simulink model "r2_2f_4x_4a_4k_r366"  (R2012b)
(part 3 of 114)

      mask prompts: storage "Storage medium"; dram_dimm "DRAM dimm"; dram_clock "DRAM clock rate"; nsamples "Number of Samples (2^?)"; data_width "Data width"; offset "Start delay support"; circap "Circular capture support"; value "Extra value capture support"; use_dsp48 "Use DSP48s to implement counters"
      mask help:
      | Standard snap block, but with the following optional extras;
      |  1) Optionally delay the fabric trigger by a user-specified number of valids.
      |  2) Capture continuously after a trigger until a stop pulse is received. Data is captured into BRAM continuously, with old data being overwritten until a stop command is received. Then stop capturing when memory is filled. This enables you to get some data before and some data after the stop pulse. Use the 'tr_en_cnt' register to determine where you are in your vector. 'Addr' register's MSb now indicates 'busy capturing'.
      |  3) Optionally capture a value on an input port to a register at the same time as the first data sample.
      |  4) Implement counters using DSP48Es to save resources.
      mask init: same as r2_2f_4x_4a_4k_r366/snap_vacc0
      mask TypeOptions storage: bram | dram
      mask Callback storage: snapshot_callback();
      mask TypeOptions dram_dimm: 1 | 2 | 3 | 4
      mask TypeOptions dram_clock: 200 | 250 | 266 | 300 | 333
      mask TypeOptions data_width: 8 | 16 | 32 | 64 | 128
  snap_xeng2 : Subsystem  Tag=casper:snapshot  AncestorBlock=casper_library_scopes/snapshot  mask(snapshot){storage=bram, dram_dimm=1, dram_clock=200, nsamples=11, data_width=32, offset=on, circap=off, value=off, use_dsp48=on}
      mask prompts: storage "Storage medium"; dram_dimm "DRAM dimm"; dram_clock "DRAM clock rate"; nsamples "Number of Samples (2^?)"; data_width "Data width"; offset "Start delay support"; circap "Circular capture support"; value "Extra value capture support"; use_dsp48 "Use DSP48s to implement counters"
      mask help:
      | Standard snap block, but with the following optional extras;
      |  1) Optionally delay the fabric trigger by a user-specified number of valids.
      |  2) Capture continuously after a trigger until a stop pulse is received. Data is captured into BRAM continuously, with old data being overwritten until a stop command is received. Then stop capturing when memory is filled. This enables you to get some data before and some data after the stop pulse. Use the 'tr_en_cnt' register to determine where you are in your vector. 'Addr' register's MSb now indicates 'busy capturing'.
      |  3) Optionally capture a value on an input port to a register at the same time as the first data sample.
      |  4) Implement counters using DSP48Es to save resources.
      mask init: same as r2_2f_4x_4a_4k_r366/snap_vacc0
      mask TypeOptions storage: bram | dram
      mask Callback storage: snapshot_callback();
      mask TypeOptions dram_dimm: 1 | 2 | 3 | 4
      mask TypeOptions dram_clock: 200 | 250 | 266 | 300 | 333
      mask TypeOptions data_width: 8 | 16 | 32 | 64 | 128
  snap_xeng3 : Subsystem  Tag=casper:snapshot  AncestorBlock=casper_library_scopes/snapshot  mask(snapshot){storage=bram, dram_dimm=1, dram_clock=200, nsamples=11, data_width=32, offset=on, circap=off, value=off, use_dsp48=on}
      mask prompts: storage "Storage medium"; dram_dimm "DRAM dimm"; dram_clock "DRAM clock rate"; nsamples "Number of Samples (2^?)"; data_width "Data width"; offset "Start delay support"; circap "Circular capture support"; value "Extra value capture support"; use_dsp48 "Use DSP48s to implement counters"
      mask help:
      | Standard snap block, but with the following optional extras;
      |  1) Optionally delay the fabric trigger by a user-specified number of valids.
      |  2) Capture continuously after a trigger until a stop pulse is received. Data is captured into BRAM continuously, with old data being overwritten until a stop command is received. Then stop capturing when memory is filled. This enables you to get some data before and some data after the stop pulse. Use the 'tr_en_cnt' register to determine where you are in your vector. 'Addr' register's MSb now indicates 'busy capturing'.
      |  3) Optionally capture a value on an input port to a register at the same time as the first data sample.
      |  4) Implement counters using DSP48Es to save resources.
      mask init: same as r2_2f_4x_4a_4k_r366/snap_vacc0
      mask TypeOptions storage: bram | dram
      mask Callback storage: snapshot_callback();
      mask TypeOptions dram_dimm: 1 | 2 | 3 | 4
      mask TypeOptions dram_clock: 200 | 250 | 266 | 300 | 333
      mask TypeOptions data_width: 8 | 16 | 32 | 64 | 128
  spead_unpack0 : Subsystem  Tag=casper:spead_unpack  AncestorBlock=casper_library_communications/spead_unpack  mask(spead_unpack_mask){payload_length=128, header_ids=[hex2dec('1600'),hex2dec('4101'),hex2dec('4102'), hex2dec('4103')], spead_msw=64, spead_lsw=48, spead_version=4, combine_errors=on}
      mask prompts: payload_length "Payload length in 64-bit words"; header_ids "SPEAD header IDs (decimal)"; spead_msw "SPEAD Flavour (MSw)"; spead_lsw "SPEAD Flavour (LSw)"; spead_version "SPEAD version"; combine_errors "Combine error flags"
      mask help: This block receives a 64-bit-word stream that contains a SPEAD stream. It checks the SPEAD headers are being correctly received. It presents the user with all headers on the first valid cycle of data along with a flag to indicate a header or packet-length error.
      mask init:
      | spead_unpack_init(gcb)
  spead_unpack1 : Subsystem  Tag=casper:spead_unpack  AncestorBlock=casper_library_communications/spead_unpack  mask(spead_unpack_mask){payload_length=128, header_ids=[hex2dec('1600'),hex2dec('4101'),hex2dec('4102'), hex2dec('4103')], spead_msw=64, spead_lsw=48, spead_version=4, combine_errors=on}
      mask prompts: payload_length "Payload length in 64-bit words"; header_ids "SPEAD header IDs (decimal)"; spead_msw "SPEAD Flavour (MSw)"; spead_lsw "SPEAD Flavour (LSw)"; spead_version "SPEAD version"; combine_errors "Combine error flags"
      mask help: This block receives a 64-bit-word stream that contains a SPEAD stream. It checks the SPEAD headers are being correctly received. It presents the user with all headers on the first valid cycle of data along with a flag to indicate a header or packet-length error.
      mask init:
      | spead_unpack_init(gcb)
  status0 : Subsystem  Tag=xps:sw_reg  AncestorBlock=xps_library/software register  mask(swreg){mode=fields of equal size, io_dir=To Processor, io_delay=1, sample_period=1, names=[gbe_down rx_dest_err feng_rx_err fft_err feng_qdr_err feng_chk_err adc_over noise_diode_en vacc_err rx_bad_pkt rx_bad_frame tx_over xeng_bad_dat pack_err rxing_data txing_data], bitwidths=1, arith_types=2, bin_pts=0, sim_port=off, show_format=off}
      mask prompts: io_dir "I/O direction"; io_delay "I/O delay"; sample_period "Sample period"; names "Names [msb ... lsb]:"; bitwidths "Bitwidth:"; arith_types "Type (ufix=0, fix=1, bool=2):"; bin_pts "Binary pt:"; sim_port "Provide sim input/output?"; show_format "Print format string?"
      mask init:
      | swreg_init(gcb)
      settings: AttributesFormatString=16 outputs
      mask TypeOptions mode: one value | fields of equal size | fields of arbitrary size
      mask Callback mode: swreg_cb(gcb);
      mask TypeOptions io_dir: To Processor | From Processor
      mask Callback io_dir:
      | mask_enables = get_param(gcb, 'MaskEnables');
      | mask_names = get_param(gcb, 'MaskNames');
      | if strcmp(get_param(gcb, 'io_dir'), 'To Processor'),
      |     mask_enables{ismember(mask_names, 'sample_period')} = 'off';
      | else
      |     mask_enables{ismember(mask_names, 'sample_period')} = 'on';
      | end
      | set_param(gcb, 'MaskEnables', mask_enables);
      mask Callback bitwidths:
      | blk = gcb;
      | mode = get_param(blk, 'mode');
      | current_widths = eval(get_param(blk, 'bitwidths'));
      | if (strcmp(mode, 'one value') || strcmp(mode, 'fields of equal size')) && (length(current_widths) > 1),
      |     error('Only one width may be specified for this mode.');
      | elseif strcmp(mode, 'fields of arbitrary size')
      |     current_names = textscan(strtrim(strrep(strrep(get_param(blk, 'names'), ']', ''), '[', '')), '%s');
      |     current_names = current_names{1};
      |     numios = length(current_names);
      |     if length(current_widths) ~= numios,
      |         error('%d field names specified, but %d widths?', numios, length(current_widths));
      |     end
      | end
      | total_width = 0;
      | for ctr = 1 : length(current_widths),
      |     total_width = total_width + current_widths(ctr);
      | end
      | if total_width > 32,
      |     error('Total width must be 32 or less, set to %d.', total_width);
      | end
      mask Callback arith_types:
      | blk = gcb;
      | mode = get_param(blk, 'mode');
      | current_types = eval(get_param(blk, 'arith_types'));
      | numios = length(current_types);
      | if (strcmp(mode, 'one value') || strcmp(mode, 'fields of equal size')) && (length(current_types) > 1),
      |     error('Only one type may be specified for this mode.');
      | elseif strcmp(mode, 'fields of arbitrary size')
      |     current_names = textscan(strtrim(strrep(strrep(get_param(blk, 'names'), ']', ''), '[', '')), '%s');
      |     current_names = current_names{1};
      |     numios = length(current_names);
      |     if length(current_types) ~= numios,
      |         error('%d field names specified, but %d types?', numios, length(current_types));
      |     end
      | end
      | problem = 0;
      | for ctr = 1 : numios,
      |     t = current_types(ctr);
      |     if (t < 0) || (t > 2),
      |         problem = t;
      |         ctr = numios + 1;
      |     end
      | end
      | if problem ~= 0,
      |     error('Type cannot be %i, must be 0, 1 or 2.', problem);
      | end
      mask Callback bin_pts:
      | blk = gcb;
      | mode = get_param(blk, 'mode');
      | current_bins = eval(get_param(blk, 'bin_pts'));
      | if (strcmp(mode, 'one value') || strcmp(mode, 'fields of equal size')) && (length(current_bins) > 1),
      |     error('Only one binary pt may be specified for this mode.');
      | elseif strcmp(mode, 'fields of arbitrary size')
      |     current_names = textscan(strtrim(strrep(strrep(get_param(blk, 'names'), ']', ''), '[', '')), '%s');
      |     current_names = current_names{1};
      |     numios = length(current_names);
      |     if length(current_bins) ~= numios,
      |         error('%d field names specified, but %d binary pts?', numios, length(current_bins));
      |     end
      | end
  status1 : Subsystem  Tag=xps:sw_reg  AncestorBlock=xps_library/software register  mask(swreg){mode=fields of equal size, io_dir=To Processor, io_delay=1, sample_period=1, names=[gbe_down rx_dest_err feng_rx_err fft_err feng_qdr_err feng_chk_err adc_over noise_diode_en vacc_err rx_bad_pkt rx_bad_frame tx_over xeng_bad_dat pack_err rxing_data txing_data], bitwidths=1, arith_types=2, bin_pts=0, sim_port=off, show_format=off}
      mask prompts: io_dir "I/O direction"; io_delay "I/O delay"; sample_period "Sample period"; names "Names [msb ... lsb]:"; bitwidths "Bitwidth:"; arith_types "Type (ufix=0, fix=1, bool=2):"; bin_pts "Binary pt:"; sim_port "Provide sim input/output?"; show_format "Print format string?"
      mask init:
      | swreg_init(gcb)
      settings: AttributesFormatString=16 outputs
      mask TypeOptions mode: one value | fields of equal size | fields of arbitrary size
      mask Callback mode: swreg_cb(gcb);
      mask TypeOptions io_dir: To Processor | From Processor
      mask Callback io_dir:
      | mask_enables = get_param(gcb, 'MaskEnables');
      | mask_names = get_param(gcb, 'MaskNames');
      | if strcmp(get_param(gcb, 'io_dir'), 'To Processor'),
      |     mask_enables{ismember(mask_names, 'sample_period')} = 'off';
      | else
      |     mask_enables{ismember(mask_names, 'sample_period')} = 'on';
      | end
      | set_param(gcb, 'MaskEnables', mask_enables);
      mask Callback bitwidths:
      | blk = gcb;
      | mode = get_param(blk, 'mode');
      | current_widths = eval(get_param(blk, 'bitwidths'));
      | if (strcmp(mode, 'one value') || strcmp(mode, 'fields of equal size')) && (length(current_widths) > 1),
      |     error('Only one width may be specified for this mode.');
      | elseif strcmp(mode, 'fields of arbitrary size')
      |     current_names = textscan(strtrim(strrep(strrep(get_param(blk, 'names'), ']', ''), '[', '')), '%s');
      |     current_names = current_names{1};
      |     numios = length(current_names);
      |     if length(current_widths) ~= numios,
      |         error('%d field names specified, but %d widths?', numios, length(current_widths));
      |     end
      | end
      | total_width = 0;
      | for ctr = 1 : length(current_widths),
      |     total_width = total_width + current_widths(ctr);
      | end
      | if total_width > 32,
      |     error('Total width must be 32 or less, set to %d.', total_width);
      | end
      mask Callback arith_types:
      | blk = gcb;
      | mode = get_param(blk, 'mode');
      | current_types = eval(get_param(blk, 'arith_types'));
      | numios = length(current_types);
      | if (strcmp(mode, 'one value') || strcmp(mode, 'fields of equal size')) && (length(current_types) > 1),
      |     error('Only one type may be specified for this mode.');
      | elseif strcmp(mode, 'fields of arbitrary size')
      |     current_names = textscan(strtrim(strrep(strrep(get_param(blk, 'names'), ']', ''), '[', '')), '%s');
      |     current_names = current_names{1};
      |     numios = length(current_names);
      |     if length(current_types) ~= numios,
      |         error('%d field names specified, but %d types?', numios, length(current_types));
      |     end
      | end
      | problem = 0;
      | for ctr = 1 : numios,
      |     t = current_types(ctr);
      |     if (t < 0) || (t > 2),
      |         problem = t;
      |         ctr = numios + 1;
      |     end
      | end
      | if problem ~= 0,
      |     error('Type cannot be %i, must be 0, 1 or 2.', problem);
      | end
      mask Callback bin_pts:
      | blk = gcb;
      | mode = get_param(blk, 'mode');
      | current_bins = eval(get_param(blk, 'bin_pts'));
      | if (strcmp(mode, 'one value') || strcmp(mode, 'fields of equal size')) && (length(current_bins) > 1),
      |     error('Only one binary pt may be specified for this mode.');
      | elseif strcmp(mode, 'fields of arbitrary size')
      |     current_names = textscan(strtrim(strrep(strrep(get_param(blk, 'names'), ']', ''), '[', '')), '%s');
      |     current_names = current_names{1};
      |     numios = length(current_names);
      |     if length(current_bins) ~= numios,
      |         error('%d field names specified, but %d binary pts?', numios, length(current_bins));
      |     end
      | end
  status2 : Subsystem  Tag=xps:sw_reg  AncestorBlock=xps_library/software register  mask(swreg){mode=fields of equal size, io_dir=To Processor, io_delay=1, sample_period=1, names=[gbe_down rx_dest_err feng_rx_err fft_err feng_qdr_err feng_chk_err adc_over noise_diode_en vacc_err rx_bad_pkt rx_bad_frame tx_over xeng_bad_dat pack_err rxing_data txing_data], bitwidths=1, arith_types=2, bin_pts=0, sim_port=off, show_format=off}
      mask prompts: io_dir "I/O direction"; io_delay "I/O delay"; sample_period "Sample period"; names "Names [msb ... lsb]:"; bitwidths "Bitwidth:"; arith_types "Type (ufix=0, fix=1, bool=2):"; bin_pts "Binary pt:"; sim_port "Provide sim input/output?"; show_format "Print format string?"
      mask init:
      | swreg_init(gcb)
      settings: AttributesFormatString=16 outputs
      mask TypeOptions mode: one value | fields of equal size | fields of arbitrary size
      mask Callback mode: swreg_cb(gcb);
      mask TypeOptions io_dir: To Processor | From Processor
      mask Callback io_dir:
      | mask_enables = get_param(gcb, 'MaskEnables');
      | mask_names = get_param(gcb, 'MaskNames');
      | if strcmp(get_param(gcb, 'io_dir'), 'To Processor'),
      |     mask_enables{ismember(mask_names, 'sample_period')} = 'off';
      | else
      |     mask_enables{ismember(mask_names, 'sample_period')} = 'on';
      | end
      | set_param(gcb, 'MaskEnables', mask_enables);
      mask Callback bitwidths:
      | blk = gcb;
      | mode = get_param(blk, 'mode');
      | current_widths = eval(get_param(blk, 'bitwidths'));
      | if (strcmp(mode, 'one value') || strcmp(mode, 'fields of equal size')) && (length(current_widths) > 1),
      |     error('Only one width may be specified for this mode.');
      | elseif strcmp(mode, 'fields of arbitrary size')
      |     current_names = textscan(strtrim(strrep(strrep(get_param(blk, 'names'), ']', ''), '[', '')), '%s');
      |     current_names = current_names{1};
      |     numios = length(current_names);
      |     if length(current_widths) ~= numios,
      |         error('%d field names specified, but %d widths?', numios, length(current_widths));
      |     end
      | end
      | total_width = 0;
      | for ctr = 1 : length(current_widths),
      |     total_width = total_width + current_widths(ctr);
      | end
      | if total_width > 32,
      |     error('Total width must be 32 or less, set to %d.', total_width);
      | end
      mask Callback arith_types:
      | blk = gcb;
      | mode = get_param(blk, 'mode');
      | current_types = eval(get_param(blk, 'arith_types'));
      | numios = length(current_types);
      | if (strcmp(mode, 'one value') || strcmp(mode, 'fields of equal size')) && (length(current_types) > 1),
      |     error('Only one type may be specified for this mode.');
      | elseif strcmp(mode, 'fields of arbitrary size')
      |     current_names = textscan(strtrim(strrep(strrep(get_param(blk, 'names'), ']', ''), '[', '')), '%s');
      |     current_names = current_names{1};
      |     numios = length(current_names);
      |     if length(current_types) ~= numios,
      |         error('%d field names specified, but %d types?', numios, length(current_types));
      |     end
      | end
      | problem = 0;
      | for ctr = 1 : numios,
      |     t = current_types(ctr);
      |     if (t < 0) || (t > 2),
      |         problem = t;
      |         ctr = numios + 1;
      |     end
      | end
      | if problem ~= 0,
      |     error('Type cannot be %i, must be 0, 1 or 2.', problem);
      | end
      mask Callback bin_pts:
      | blk = gcb;
      | mode = get_param(blk, 'mode');
      | current_bins = eval(get_param(blk, 'bin_pts'));
      | if (strcmp(mode, 'one value') || strcmp(mode, 'fields of equal size')) && (length(current_bins) > 1),
      |     error('Only one binary pt may be specified for this mode.');
      | elseif strcmp(mode, 'fields of arbitrary size')
      |     current_names = textscan(strtrim(strrep(strrep(get_param(blk, 'names'), ']', ''), '[', '')), '%s');
      |     current_names = current_names{1};
      |     numios = length(current_names);
      |     if length(current_bins) ~= numios,
      |         error('%d field names specified, but %d binary pts?', numios, length(current_bins));
      |     end
      | end
  status3 : Subsystem  Tag=xps:sw_reg  AncestorBlock=xps_library/software register  mask(swreg){mode=fields of equal size, io_dir=To Processor, io_delay=1, sample_period=1, names=[gbe_down rx_dest_err feng_rx_err fft_err feng_qdr_err feng_chk_err adc_over noise_diode_en vacc_err rx_bad_pkt rx_bad_frame tx_over xeng_bad_dat pack_err rxing_data txing_data], bitwidths=1, arith_types=2, bin_pts=0, sim_port=off, show_format=off}
      mask prompts: io_dir "I/O direction"; io_delay "I/O delay"; sample_period "Sample period"; names "Names [msb ... lsb]:"; bitwidths "Bitwidth:"; arith_types "Type (ufix=0, fix=1, bool=2):"; bin_pts "Binary pt:"; sim_port "Provide sim input/output?"; show_format "Print format string?"
      mask init:
      | swreg_init(gcb)
      settings: AttributesFormatString=16 outputs
      mask TypeOptions mode: one value | fields of equal size | fields of arbitrary size
      mask Callback mode: swreg_cb(gcb);
      mask TypeOptions io_dir: To Processor | From Processor
      mask Callback io_dir:
      | mask_enables = get_param(gcb, 'MaskEnables');
      | mask_names = get_param(gcb, 'MaskNames');
      | if strcmp(get_param(gcb, 'io_dir'), 'To Processor'),
      |     mask_enables{ismember(mask_names, 'sample_period')} = 'off';
      | else
      |     mask_enables{ismember(mask_names, 'sample_period')} = 'on';
      | end
      | set_param(gcb, 'MaskEnables', mask_enables);
      mask Callback bitwidths:
      | blk = gcb;
      | mode = get_param(blk, 'mode');
      | current_widths = eval(get_param(blk, 'bitwidths'));
      | if (strcmp(mode, 'one value') || strcmp(mode, 'fields of equal size')) && (length(current_widths) > 1),
      |     error('Only one width may be specified for this mode.');
      | elseif strcmp(mode, 'fields of arbitrary size')
      |     current_names = textscan(strtrim(strrep(strrep(get_param(blk, 'names'), ']', ''), '[', '')), '%s');
      |     current_names = current_names{1};
      |     numios = length(current_names);
      |     if length(current_widths) ~= numios,
      |         error('%d field names specified, but %d widths?', numios, length(current_widths));
      |     end
      | end
      | total_width = 0;
      | for ctr = 1 : length(current_widths),
      |     total_width = total_width + current_widths(ctr);
      | end
      | if total_width > 32,
      |     error('Total width must be 32 or less, set to %d.', total_width);
      | end
      mask Callback arith_types:
      | blk = gcb;
      | mode = get_param(blk, 'mode');
      | current_types = eval(get_param(blk, 'arith_types'));
      | numios = length(current_types);
      | if (strcmp(mode, 'one value') || strcmp(mode, 'fields of equal size')) && (length(current_types) > 1),
      |     error('Only one type may be specified for this mode.');
      | elseif strcmp(mode, 'fields of arbitrary size')
      |     current_names = textscan(strtrim(strrep(strrep(get_param(blk, 'names'), ']', ''), '[', '')), '%s');
      |     current_names = current_names{1};
      |     numios = length(current_names);
      |     if length(current_types) ~= numios,
      |         error('%d field names specified, but %d types?', numios, length(current_types));
      |     end
      | end
      | problem = 0;
      | for ctr = 1 : numios,
      |     t = current_types(ctr);
      |     if (t < 0) || (t > 2),
      |         problem = t;
      |         ctr = numios + 1;
      |     end
      | end
      | if problem ~= 0,
      |     error('Type cannot be %i, must be 0, 1 or 2.', problem);
      | end
      mask Callback bin_pts:
      | blk = gcb;
      | mode = get_param(blk, 'mode');
      | current_bins = eval(get_param(blk, 'bin_pts'));
      | if (strcmp(mode, 'one value') || strcmp(mode, 'fields of equal size')) && (length(current_bins) > 1),
      |     error('Only one binary pt may be specified for this mode.');
      | elseif strcmp(mode, 'fields of arbitrary size')
      |     current_names = textscan(strtrim(strrep(strrep(get_param(blk, 'names'), ']', ''), '[', '')), '%s');
      |     current_names = current_names{1};
      |     numios = length(current_names);
      |     if length(current_bins) ~= numios,
      |         error('%d field names specified, but %d binary pts?', numios, length(current_bins));
      |     end
      | end
  tvg_sel : Subsystem  Tag=xps:sw_reg  AncestorBlock=xps_library/software register  mask(swreg){mode=fields of arbitrary size, io_dir=From Processor, io_delay=1, sample_period=1, names=[xaui descr xeng vacc], bitwidths=[1 2 2 6], arith_types=[0 0 0 0], bin_pts=[0 0 0 0], sim_port=off, show_format=off}
      mask prompts: io_dir "I/O direction"; io_delay "I/O delay"; sample_period "Sample period"; names "Names [msb ... lsb]:"; bitwidths "Bitwidths [msb ... lsb]:"; arith_types "Types (ufix=0, fix=1, bool=2) [msb ... lsb]:"; bin_pts "Binary pts [msb ... lsb]:"; sim_port "Provide sim input/output?"; show_format "Print format string?"
      mask init:
      | swreg_init(gcb)
      settings: AttributesFormatString=4 inputs
      mask TypeOptions mode: one value | fields of equal size | fields of arbitrary size
      mask Callback mode: swreg_cb(gcb);
      mask TypeOptions io_dir: To Processor | From Processor
      mask Callback io_dir:
      | mask_enables = get_param(gcb, 'MaskEnables');
      | mask_names = get_param(gcb, 'MaskNames');
      | if strcmp(get_param(gcb, 'io_dir'), 'To Processor'),
      |     mask_enables{ismember(mask_names, 'sample_period')} = 'off';
      | else
      |     mask_enables{ismember(mask_names, 'sample_period')} = 'on';
      | end
      | set_param(gcb, 'MaskEnables', mask_enables);
      mask Callback bitwidths:
      | blk = gcb;
      | mode = get_param(blk, 'mode');
      | current_widths = eval(get_param(blk, 'bitwidths'));
      | if (strcmp(mode, 'one value') || strcmp(mode, 'fields of equal size')) && (length(current_widths) > 1),
      |     error('Only one width may be specified for this mode.');
      | elseif strcmp(mode, 'fields of arbitrary size')
      |     current_names = textscan(strtrim(strrep(strrep(get_param(blk, 'names'), ']', ''), '[', '')), '%s');
      |     current_names = current_names{1};
      |     numios = length(current_names);
      |     if length(current_widths) ~= numios,
      |         error('%d field names specified, but %d widths?', numios, length(current_widths));
      |     end
      | end
      | total_width = 0;
      | for ctr = 1 : length(current_widths),
      |     total_width = total_width + current_widths(ctr);
      | end
      | if total_width > 32,
      |     error('Total width must be 32 or less, set to %d.', total_width);
      | end
      mask Callback arith_types:
      | blk = gcb;
      | mode = get_param(blk, 'mode');
      | current_types = eval(get_param(blk, 'arith_types'));
      | numios = length(current_types);
      | if (strcmp(mode, 'one value') || strcmp(mode, 'fields of equal size')) && (length(current_types) > 1),
      |     error('Only one type may be specified for this mode.');
      | elseif strcmp(mode, 'fields of arbitrary size')
      |     current_names = textscan(strtrim(strrep(strrep(get_param(blk, 'names'), ']', ''), '[', '')), '%s');
      |     current_names = current_names{1};
      |     numios = length(current_names);
      |     if length(current_types) ~= numios,
      |         error('%d field names specified, but %d types?', numios, length(current_types));
      |     end
      | end
      | problem = 0;
      | for ctr = 1 : numios,
      |     t = current_types(ctr);
      |     if (t < 0) || (t > 2),
      |         problem = t;
      |         ctr = numios + 1;
      |     end
      | end
      | if problem ~= 0,
      |     error('Type cannot be %i, must be 0, 1 or 2.', problem);
      | end
      mask Callback bin_pts:
      | blk = gcb;
      | mode = get_param(blk, 'mode');
      | current_bins = eval(get_param(blk, 'bin_pts'));
      | if (strcmp(mode, 'one value') || strcmp(mode, 'fields of equal size')) && (length(current_bins) > 1),
      |     error('Only one binary pt may be specified for this mode.');
      | elseif strcmp(mode, 'fields of arbitrary size')
      |     current_names = textscan(strtrim(strrep(strrep(get_param(blk, 'names'), ']', ''), '[', '')), '%s');
      |     current_names = current_names{1};
      |     numios = length(current_names);
      |     if length(current_bins) ~= numios,
      |         error('%d field names specified, but %d binary pts?', numios, length(current_bins));
      |     end
      | end
  txip : Subsystem  Tag=xps:sw_reg  AncestorBlock=xps_library/software register  mask(swreg){mode=one value, io_dir=From Processor, io_delay=1, sample_period=1, names=txip, bitwidths=32, arith_types=0, bin_pts=0, sim_port=off, show_format=off}
      mask prompts: io_dir "I/O direction"; io_delay "I/O delay"; sample_period "Sample period"; names "Name:"; bitwidths "Bitwidth:"; arith_types "Type (ufix=0, fix=1, bool=2):"; bin_pts "Binary pt:"; sim_port "Provide sim input/output?"; show_format "Print format string?"
      mask init:
      | swreg_init(gcb)
      settings: AttributesFormatString=1input
      mask TypeOptions mode: one value | fields of equal size | fields of arbitrary size
      mask Callback mode: swreg_cb(gcb);
      mask TypeOptions io_dir: To Processor | From Processor
      mask Callback io_dir:
      | mask_enables = get_param(gcb, 'MaskEnables');
      | mask_names = get_param(gcb, 'MaskNames');
      | if strcmp(get_param(gcb, 'io_dir'), 'To Processor'),
      |     mask_enables{ismember(mask_names, 'sample_period')} = 'off';
      | else
      |     mask_enables{ismember(mask_names, 'sample_period')} = 'on';
      | end
      | set_param(gcb, 'MaskEnables', mask_enables);
      mask Callback bitwidths:
      | blk = gcb;
      | mode = get_param(blk, 'mode');
      | current_widths = eval(get_param(blk, 'bitwidths'));
      | if (strcmp(mode, 'one value') || strcmp(mode, 'fields of equal size')) && (length(current_widths) > 1),
      |     error('Only one width may be specified for this mode.');
      | elseif strcmp(mode, 'fields of arbitrary size')
      |     current_names = textscan(strtrim(strrep(strrep(get_param(blk, 'names'), ']', ''), '[', '')), '%s');
      |     current_names = current_names{1};
      |     numios = length(current_names);
      |     if length(current_widths) ~= numios,
      |         error('%d field names specified, but %d widths?', numios, length(current_widths));
      |     end
      | end
      | total_width = 0;
      | for ctr = 1 : length(current_widths),
      |     total_width = total_width + current_widths(ctr);
      | end
      | if total_width > 32,
      |     error('Total width must be 32 or less, set to %d.', total_width);
      | end
      mask Callback arith_types:
      | blk = gcb;
      | mode = get_param(blk, 'mode');
      | current_types = eval(get_param(blk, 'arith_types'));
      | numios = length(current_types);
      | if (strcmp(mode, 'one value') || strcmp(mode, 'fields of equal size')) && (length(current_types) > 1),
      |     error('Only one type may be specified for this mode.');
      | elseif strcmp(mode, 'fields of arbitrary size')
      |     current_names = textscan(strtrim(strrep(strrep(get_param(blk, 'names'), ']', ''), '[', '')), '%s');
      |     current_names = current_names{1};
      |     numios = length(current_names);
      |     if length(current_types) ~= numios,
      |         error('%d field names specified, but %d types?', numios, length(current_types));
      |     end
      | end
      | problem = 0;
      | for ctr = 1 : numios,
      |     t = current_types(ctr);
      |     if (t < 0) || (t > 2),
      |         problem = t;
      |         ctr = numios + 1;
      |     end
      | end
      | if problem ~= 0,
      |     error('Type cannot be %i, must be 0, 1 or 2.', problem);
      | end
      mask Callback bin_pts:
      | blk = gcb;
      | mode = get_param(blk, 'mode');
      | current_bins = eval(get_param(blk, 'bin_pts'));
      | if (strcmp(mode, 'one value') || strcmp(mode, 'fields of equal size')) && (length(current_bins) > 1),
      |     error('Only one binary pt may be specified for this mode.');
      | elseif strcmp(mode, 'fields of arbitrary size')
      |     current_names = textscan(strtrim(strrep(strrep(get_param(blk, 'names'), ']', ''), '[', '')), '%s');
      |     current_names = current_names{1};
      |     numios = length(current_names);
      |     if length(current_bins) ~= numios,
      |         error('%d field names specified, but %d binary pts?', numios, length(current_bins));
      |     end
      | end
  txport : Subsystem  Tag=xps:sw_reg  AncestorBlock=xps_library/software register  mask(swreg){mode=one value, io_dir=From Processor, io_delay=1, sample_period=1, names=txport, bitwidths=32, arith_types=0, bin_pts=0, sim_port=off, show_format=off}
      mask prompts: io_dir "I/O direction"; io_delay "I/O delay"; sample_period "Sample period"; names "Name:"; bitwidths "Bitwidth:"; arith_types "Type (ufix=0, fix=1, bool=2):"; bin_pts "Binary pt:"; sim_port "Provide sim input/output?"; show_format "Print format string?"
      mask init:
      | swreg_init(gcb)
      settings: AttributesFormatString=1input
      mask TypeOptions mode: one value | fields of equal size | fields of arbitrary size
      mask Callback mode: swreg_cb(gcb);
      mask TypeOptions io_dir: To Processor | From Processor
      mask Callback io_dir:
      | mask_enables = get_param(gcb, 'MaskEnables');
      | mask_names = get_param(gcb, 'MaskNames');
      | if strcmp(get_param(gcb, 'io_dir'), 'To Processor'),
      |     mask_enables{ismember(mask_names, 'sample_period')} = 'off';
      | else
      |     mask_enables{ismember(mask_names, 'sample_period')} = 'on';
      | end
      | set_param(gcb, 'MaskEnables', mask_enables);
      mask Callback bitwidths:
      | blk = gcb;
      | mode = get_param(blk, 'mode');
      | current_widths = eval(get_param(blk, 'bitwidths'));
      | if (strcmp(mode, 'one value') || strcmp(mode, 'fields of equal size')) && (length(current_widths) > 1),
      |     error('Only one width may be specified for this mode.');
      | elseif strcmp(mode, 'fields of arbitrary size')
      |     current_names = textscan(strtrim(strrep(strrep(get_param(blk, 'names'), ']', ''), '[', '')), '%s');
      |     current_names = current_names{1};
      |     numios = length(current_names);
      |     if length(current_widths) ~= numios,
      |         error('%d field names specified, but %d widths?', numios, length(current_widths));
      |     end
      | end
      | total_width = 0;
      | for ctr = 1 : length(current_widths),
      |     total_width = total_width + current_widths(ctr);
      | end
      | if total_width > 32,
      |     error('Total width must be 32 or less, set to %d.', total_width);
      | end
      mask Callback arith_types:
      | blk = gcb;
      | mode = get_param(blk, 'mode');
      | current_types = eval(get_param(blk, 'arith_types'));
      | numios = length(current_types);
      | if (strcmp(mode, 'one value') || strcmp(mode, 'fields of equal size')) && (length(current_types) > 1),
      |     error('Only one type may be specified for this mode.');
      | elseif strcmp(mode, 'fields of arbitrary size')
      |     current_names = textscan(strtrim(strrep(strrep(get_param(blk, 'names'), ']', ''), '[', '')), '%s');
      |     current_names = current_names{1};
      |     numios = length(current_names);
      |     if length(current_types) ~= numios,
      |         error('%d field names specified, but %d types?', numios, length(current_types));
      |     end
      | end
      | problem = 0;
      | for ctr = 1 : numios,
      |     t = current_types(ctr);
      |     if (t < 0) || (t > 2),
      |         problem = t;
      |         ctr = numios + 1;
      |     end
      | end
      | if problem ~= 0,
      |     error('Type cannot be %i, must be 0, 1 or 2.', problem);
      | end
      mask Callback bin_pts:
      | blk = gcb;
      | mode = get_param(blk, 'mode');
      | current_bins = eval(get_param(blk, 'bin_pts'));
      | if (strcmp(mode, 'one value') || strcmp(mode, 'fields of equal size')) && (length(current_bins) > 1),
      |     error('Only one binary pt may be specified for this mode.');
      | elseif strcmp(mode, 'fields of arbitrary size')
      |     current_names = textscan(strtrim(strrep(strrep(get_param(blk, 'names'), ']', ''), '[', '')), '%s');
      |     current_names = current_names{1};
      |     numios = length(current_names);
      |     if length(current_bins) ~= numios,
      |         error('%d field names specified, but %d binary pts?', numios, length(current_bins));
      |     end
      | end
  vacc_cnt0 : Subsystem  Tag=xps:sw_reg  AncestorBlock=xps_library/software register  mask(swreg){mode=one value, io_dir=To Processor, io_delay=1, sample_period=1, names=reg, bitwidths=32, arith_types=0, bin_pts=0, sim_port=off, show_format=off}
      mask prompts: io_dir "I/O direction"; io_delay "I/O delay"; sample_period "Sample period"; names "Name:"; bitwidths "Bitwidth:"; arith_types "Type (ufix=0, fix=1, bool=2):"; bin_pts "Binary pt:"; sim_port "Provide sim input/output?"; show_format "Print format string?"
      mask init:
      | swreg_init(gcb)
      settings: AttributesFormatString=1output
      mask TypeOptions mode: one value | fields of equal size | fields of arbitrary size
      mask Callback mode: swreg_cb(gcb);
      mask TypeOptions io_dir: To Processor | From Processor
      mask Callback io_dir:
      | mask_enables = get_param(gcb, 'MaskEnables');
      | mask_names = get_param(gcb, 'MaskNames');
      | if strcmp(get_param(gcb, 'io_dir'), 'To Processor'),
      |     mask_enables{ismember(mask_names, 'sample_period')} = 'off';
      | else
      |     mask_enables{ismember(mask_names, 'sample_period')} = 'on';
      | end
      | set_param(gcb, 'MaskEnables', mask_enables);
      mask Callback bitwidths:
      | blk = gcb;
      | mode = get_param(blk, 'mode');
      | current_widths = eval(get_param(blk, 'bitwidths'));
      | if (strcmp(mode, 'one value') || strcmp(mode, 'fields of equal size')) && (length(current_widths) > 1),
      |     error('Only one width may be specified for this mode.');
      | elseif strcmp(mode, 'fields of arbitrary size')
      |     current_names = textscan(strtrim(strrep(strrep(get_param(blk, 'names'), ']', ''), '[', '')), '%s');
      |     current_names = current_names{1};
      |     numios = length(current_names);
      |     if length(current_widths) ~= numios,
      |         error('%d field names specified, but %d widths?', numios, length(current_widths));
      |     end
      | end
      | total_width = 0;
      | for ctr = 1 : length(current_widths),
      |     total_width = total_width + current_widths(ctr);
      | end
      | if total_width > 32,
      |     error('Total width must be 32 or less, set to %d.', total_width);
      | end
      mask Callback arith_types:
      | blk = gcb;
      | mode = get_param(blk, 'mode');
      | current_types = eval(get_param(blk, 'arith_types'));
      | numios = length(current_types);
      | if (strcmp(mode, 'one value') || strcmp(mode, 'fields of equal size')) && (length(current_types) > 1),
      |     error('Only one type may be specified for this mode.');
      | elseif strcmp(mode, 'fields of arbitrary size')
      |     current_names = textscan(strtrim(strrep(strrep(get_param(blk, 'names'), ']', ''), '[', '')), '%s');
      |     current_names = current_names{1};
      |     numios = length(current_names);
      |     if length(current_types) ~= numios,
      |         error('%d field names specified, but %d types?', numios, length(current_types));
      |     end
      | end
      | problem = 0;
      | for ctr = 1 : numios,
      |     t = current_types(ctr);
      |     if (t < 0) || (t > 2),
      |         problem = t;
      |         ctr = numios + 1;
      |     end
      | end
      | if problem ~= 0,
      |     error('Type cannot be %i, must be 0, 1 or 2.', problem);
      | end
      mask Callback bin_pts:
      | blk = gcb;
      | mode = get_param(blk, 'mode');
      | current_bins = eval(get_param(blk, 'bin_pts'));
      | if (strcmp(mode, 'one value') || strcmp(mode, 'fields of equal size')) && (length(current_bins) > 1),
      |     error('Only one binary pt may be specified for this mode.');
      | elseif strcmp(mode, 'fields of arbitrary size')
      |     current_names = textscan(strtrim(strrep(strrep(get_param(blk, 'names'), ']', ''), '[', '')), '%s');
      |     current_names = current_names{1};
      |     numios = length(current_names);
      |     if length(current_bins) ~= numios,
      |         error('%d field names specified, but %d binary pts?', numios, length(current_bins));
      |     end
      | end
  vacc_cnt1 : Subsystem  Tag=xps:sw_reg  AncestorBlock=xps_library/software register  mask(swreg){mode=one value, io_dir=To Processor, io_delay=1, sample_period=1, names=reg, bitwidths=32, arith_types=0, bin_pts=0, sim_port=off, show_format=off}
      mask prompts: io_dir "I/O direction"; io_delay "I/O delay"; sample_period "Sample period"; names "Name:"; bitwidths "Bitwidth:"; arith_types "Type (ufix=0, fix=1, bool=2):"; bin_pts "Binary pt:"; sim_port "Provide sim input/output?"; show_format "Print format string?"
      mask init:
      | swreg_init(gcb)
      settings: AttributesFormatString=1output
      mask TypeOptions mode: one value | fields of equal size | fields of arbitrary size
      mask Callback mode: swreg_cb(gcb);
      mask TypeOptions io_dir: To Processor | From Processor
      mask Callback io_dir:
      | mask_enables = get_param(gcb, 'MaskEnables');
      | mask_names = get_param(gcb, 'MaskNames');
      | if strcmp(get_param(gcb, 'io_dir'), 'To Processor'),
      |     mask_enables{ismember(mask_names, 'sample_period')} = 'off';
      | else
      |     mask_enables{ismember(mask_names, 'sample_period')} = 'on';
      | end
      | set_param(gcb, 'MaskEnables', mask_enables);
      mask Callback bitwidths:
      | blk = gcb;
      | mode = get_param(blk, 'mode');
      | current_widths = eval(get_param(blk, 'bitwidths'));
      | if (strcmp(mode, 'one value') || strcmp(mode, 'fields of equal size')) && (length(current_widths) > 1),
      |     error('Only one width may be specified for this mode.');
      | elseif strcmp(mode, 'fields of arbitrary size')
      |     current_names = textscan(strtrim(strrep(strrep(get_param(blk, 'names'), ']', ''), '[', '')), '%s');
      |     current_names = current_names{1};
      |     numios = length(current_names);
      |     if length(current_widths) ~= numios,
      |         error('%d field names specified, but %d widths?', numios, length(current_widths));
      |     end
      | end
      | total_width = 0;
      | for ctr = 1 : length(current_widths),
      |     total_width = total_width + current_widths(ctr);
      | end
      | if total_width > 32,
      |     error('Total width must be 32 or less, set to %d.', total_width);
      | end
      mask Callback arith_types:
      | blk = gcb;
      | mode = get_param(blk, 'mode');
      | current_types = eval(get_param(blk, 'arith_types'));
      | numios = length(current_types);
      | if (strcmp(mode, 'one value') || strcmp(mode, 'fields of equal size')) && (length(current_types) > 1),
      |     error('Only one type may be specified for this mode.');
      | elseif strcmp(mode, 'fields of arbitrary size')
      |     current_names = textscan(strtrim(strrep(strrep(get_param(blk, 'names'), ']', ''), '[', '')), '%s');
      |     current_names = current_names{1};
      |     numios = length(current_names);
      |     if length(current_types) ~= numios,
      |         error('%d field names specified, but %d types?', numios, length(current_types));
      |     end
      | end
      | problem = 0;
      | for ctr = 1 : numios,
      |     t = current_types(ctr);
      |     if (t < 0) || (t > 2),
      |         problem = t;
      |         ctr = numios + 1;
      |     end
      | end
      | if problem ~= 0,
      |     error('Type cannot be %i, must be 0, 1 or 2.', problem);
      | end
      mask Callback bin_pts:
      | blk = gcb;
      | mode = get_param(blk, 'mode');
      | current_bins = eval(get_param(blk, 'bin_pts'));
      | if (strcmp(mode, 'one value') || strcmp(mode, 'fields of equal size')) && (length(current_bins) > 1),
      |     error('Only one binary pt may be specified for this mode.');
      | elseif strcmp(mode, 'fields of arbitrary size')
      |     current_names = textscan(strtrim(strrep(strrep(get_param(blk, 'names'), ']', ''), '[', '')), '%s');
      |     current_names = current_names{1};
      |     numios = length(current_names);
      |     if length(current_bins) ~= numios,
      |         error('%d field names specified, but %d binary pts?', numios, length(current_bins));
      |     end
      | end
  vacc_cnt2 : Subsystem  Tag=xps:sw_reg  AncestorBlock=xps_library/software register  mask(swreg){mode=one value, io_dir=To Processor, io_delay=1, sample_period=1, names=reg, bitwidths=32, arith_types=0, bin_pts=0, sim_port=off, show_format=off}
      mask prompts: io_dir "I/O direction"; io_delay "I/O delay"; sample_period "Sample period"; names "Name:"; bitwidths "Bitwidth:"; arith_types "Type (ufix=0, fix=1, bool=2):"; bin_pts "Binary pt:"; sim_port "Provide sim input/output?"; show_format "Print format string?"
      mask init:
      | swreg_init(gcb)
      settings: AttributesFormatString=1output
      mask TypeOptions mode: one value | fields of equal size | fields of arbitrary size
      mask Callback mode: swreg_cb(gcb);
      mask TypeOptions io_dir: To Processor | From Processor
      mask Callback io_dir:
      | mask_enables = get_param(gcb, 'MaskEnables');
      | mask_names = get_param(gcb, 'MaskNames');
      | if strcmp(get_param(gcb, 'io_dir'), 'To Processor'),
      |     mask_enables{ismember(mask_names, 'sample_period')} = 'off';
      | else
      |     mask_enables{ismember(mask_names, 'sample_period')} = 'on';
      | end
      | set_param(gcb, 'MaskEnables', mask_enables);
      mask Callback bitwidths:
      | blk = gcb;
      | mode = get_param(blk, 'mode');
      | current_widths = eval(get_param(blk, 'bitwidths'));
      | if (strcmp(mode, 'one value') || strcmp(mode, 'fields of equal size')) && (length(current_widths) > 1),
      |     error('Only one width may be specified for this mode.');
      | elseif strcmp(mode, 'fields of arbitrary size')
      |     current_names = textscan(strtrim(strrep(strrep(get_param(blk, 'names'), ']', ''), '[', '')), '%s');
      |     current_names = current_names{1};
      |     numios = length(current_names);
      |     if length(current_widths) ~= numios,
      |         error('%d field names specified, but %d widths?', numios, length(current_widths));
      |     end
      | end
      | total_width = 0;
      | for ctr = 1 : length(current_widths),
      |     total_width = total_width + current_widths(ctr);
      | end
      | if total_width > 32,
      |     error('Total width must be 32 or less, set to %d.', total_width);
      | end
      mask Callback arith_types:
      | blk = gcb;
      | mode = get_param(blk, 'mode');
      | current_types = eval(get_param(blk, 'arith_types'));
      | numios = length(current_types);
      | if (strcmp(mode, 'one value') || strcmp(mode, 'fields of equal size')) && (length(current_types) > 1),
      |     error('Only one type may be specified for this mode.');
      | elseif strcmp(mode, 'fields of arbitrary size')
      |     current_names = textscan(strtrim(strrep(strrep(get_param(blk, 'names'), ']', ''), '[', '')), '%s');
      |     current_names = current_names{1};
      |     numios = length(current_names);
      |     if length(current_types) ~= numios,
      |         error('%d field names specified, but %d types?', numios, length(current_types));
      |     end
      | end
      | problem = 0;
      | for ctr = 1 : numios,
      |     t = current_types(ctr);
      |     if (t < 0) || (t > 2),
      |         problem = t;
      |         ctr = numios + 1;
      |     end
      | end
      | if problem ~= 0,
      |     error('Type cannot be %i, must be 0, 1 or 2.', problem);
      | end
      mask Callback bin_pts:
      | blk = gcb;
      | mode = get_param(blk, 'mode');
      | current_bins = eval(get_param(blk, 'bin_pts'));
      | if (strcmp(mode, 'one value') || strcmp(mode, 'fields of equal size')) && (length(current_bins) > 1),
      |     error('Only one binary pt may be specified for this mode.');
      | elseif strcmp(mode, 'fields of arbitrary size')
      |     current_names = textscan(strtrim(strrep(strrep(get_param(blk, 'names'), ']', ''), '[', '')), '%s');
      |     current_names = current_names{1};
      |     numios = length(current_names);
      |     if length(current_bins) ~= numios,
      |         error('%d field names specified, but %d binary pts?', numios, length(current_bins));
      |     end
      | end
  vacc_cnt3 : Subsystem  Tag=xps:sw_reg  AncestorBlock=xps_library/software register  mask(swreg){mode=one value, io_dir=To Processor, io_delay=1, sample_period=1, names=reg, bitwidths=32, arith_types=0, bin_pts=0, sim_port=off, show_format=off}
      mask prompts: io_dir "I/O direction"; io_delay "I/O delay"; sample_period "Sample period"; names "Name:"; bitwidths "Bitwidth:"; arith_types "Type (ufix=0, fix=1, bool=2):"; bin_pts "Binary pt:"; sim_port "Provide sim input/output?"; show_format "Print format string?"
      mask init:
      | swreg_init(gcb)
      settings: AttributesFormatString=1output
      mask TypeOptions mode: one value | fields of equal size | fields of arbitrary size
      mask Callback mode: swreg_cb(gcb);
      mask TypeOptions io_dir: To Processor | From Processor
      mask Callback io_dir:
      | mask_enables = get_param(gcb, 'MaskEnables');
      | mask_names = get_param(gcb, 'MaskNames');
      | if strcmp(get_param(gcb, 'io_dir'), 'To Processor'),
      |     mask_enables{ismember(mask_names, 'sample_period')} = 'off';
      | else
      |     mask_enables{ismember(mask_names, 'sample_period')} = 'on';
      | end
      | set_param(gcb, 'MaskEnables', mask_enables);
      mask Callback bitwidths:
      | blk = gcb;
      | mode = get_param(blk, 'mode');
      | current_widths = eval(get_param(blk, 'bitwidths'));
      | if (strcmp(mode, 'one value') || strcmp(mode, 'fields of equal size')) && (length(current_widths) > 1),
      |     error('Only one width may be specified for this mode.');
      | elseif strcmp(mode, 'fields of arbitrary size')
      |     current_names = textscan(strtrim(strrep(strrep(get_param(blk, 'names'), ']', ''), '[', '')), '%s');
      |     current_names = current_names{1};
      |     numios = length(current_names);
      |     if length(current_widths) ~= numios,
      |         error('%d field names specified, but %d widths?', numios, length(current_widths));
      |     end
      | end
      | total_width = 0;
      | for ctr = 1 : length(current_widths),
      |     total_width = total_width + current_widths(ctr);
      | end
      | if total_width > 32,
      |     error('Total width must be 32 or less, set to %d.', total_width);
      | end
      mask Callback arith_types:
      | blk = gcb;
      | mode = get_param(blk, 'mode');
      | current_types = eval(get_param(blk, 'arith_types'));
      | numios = length(current_types);
      | if (strcmp(mode, 'one value') || strcmp(mode, 'fields of equal size')) && (length(current_types) > 1),
      |     error('Only one type may be specified for this mode.');
      | elseif strcmp(mode, 'fields of arbitrary size')
      |     current_names = textscan(strtrim(strrep(strrep(get_param(blk, 'names'), ']', ''), '[', '')), '%s');
      |     current_names = current_names{1};
      |     numios = length(current_names);
      |     if length(current_types) ~= numios,
      |         error('%d field names specified, but %d types?', numios, length(current_types));
      |     end
      | end
      | problem = 0;
      | for ctr = 1 : numios,
      |     t = current_types(ctr);
      |     if (t < 0) || (t > 2),
      |         problem = t;
      |         ctr = numios + 1;
      |     end
      | end
      | if problem ~= 0,
      |     error('Type cannot be %i, must be 0, 1 or 2.', problem);
      | end
      mask Callback bin_pts:
      | blk = gcb;
      | mode = get_param(blk, 'mode');
      | current_bins = eval(get_param(blk, 'bin_pts'));
      | if (strcmp(mode, 'one value') || strcmp(mode, 'fields of equal size')) && (length(current_bins) > 1),
      |     error('Only one binary pt may be specified for this mode.');
      | elseif strcmp(mode, 'fields of arbitrary size')
      |     current_names = textscan(strtrim(strrep(strrep(get_param(blk, 'names'), ']', ''), '[', '')), '%s');
      |     current_names = current_names{1};
      |     numios = length(current_names);
      |     if length(current_bins) ~= numios,
      |         error('%d field names specified, but %d binary pts?', numios, length(current_bins));
      |     end
      | end
  vacc_err_cnt0 : Subsystem  Tag=xps:sw_reg  AncestorBlock=xps_library/software register  mask(swreg){mode=one value, io_dir=To Processor, io_delay=1, sample_period=1, names=reg, bitwidths=32, arith_types=0, bin_pts=0, sim_port=off, show_format=off}
      mask prompts: io_dir "I/O direction"; io_delay "I/O delay"; sample_period "Sample period"; names "Name:"; bitwidths "Bitwidth:"; arith_types "Type (ufix=0, fix=1, bool=2):"; bin_pts "Binary pt:"; sim_port "Provide sim input/output?"; show_format "Print format string?"
      mask init:
      | swreg_init(gcb)
      settings: AttributesFormatString=1output
      mask TypeOptions mode: one value | fields of equal size | fields of arbitrary size
      mask Callback mode: swreg_cb(gcb);
      mask TypeOptions io_dir: To Processor | From Processor
      mask Callback io_dir:
      | mask_enables = get_param(gcb, 'MaskEnables');
      | mask_names = get_param(gcb, 'MaskNames');
      | if strcmp(get_param(gcb, 'io_dir'), 'To Processor'),
      |     mask_enables{ismember(mask_names, 'sample_period')} = 'off';
      | else
      |     mask_enables{ismember(mask_names, 'sample_period')} = 'on';
      | end
      | set_param(gcb, 'MaskEnables', mask_enables);
      mask Callback bitwidths:
      | blk = gcb;
      | mode = get_param(blk, 'mode');
      | current_widths = eval(get_param(blk, 'bitwidths'));
      | if (strcmp(mode, 'one value') || strcmp(mode, 'fields of equal size')) && (length(current_widths) > 1),
      |     error('Only one width may be specified for this mode.');
      | elseif strcmp(mode, 'fields of arbitrary size')
      |     current_names = textscan(strtrim(strrep(strrep(get_param(blk, 'names'), ']', ''), '[', '')), '%s');
      |     current_names = current_names{1};
      |     numios = length(current_names);
      |     if length(current_widths) ~= numios,
      |         error('%d field names specified, but %d widths?', numios, length(current_widths));
      |     end
      | end
      | total_width = 0;
      | for ctr = 1 : length(current_widths),
      |     total_width = total_width + current_widths(ctr);
      | end
      | if total_width > 32,
      |     error('Total width must be 32 or less, set to %d.', total_width);
      | end
      mask Callback arith_types:
      | blk = gcb;
      | mode = get_param(blk, 'mode');
      | current_types = eval(get_param(blk, 'arith_types'));
      | numios = length(current_types);
      | if (strcmp(mode, 'one value') || strcmp(mode, 'fields of equal size')) && (length(current_types) > 1),
      |     error('Only one type may be specified for this mode.');
      | elseif strcmp(mode, 'fields of arbitrary size')
      |     current_names = textscan(strtrim(strrep(strrep(get_param(blk, 'names'), ']', ''), '[', '')), '%s');
      |     current_names = current_names{1};
      |     numios = length(current_names);
      |     if length(current_types) ~= numios,
      |         error('%d field names specified, but %d types?', numios, length(current_types));
      |     end
      | end
      | problem = 0;
      | for ctr = 1 : numios,
      |     t = current_types(ctr);
      |     if (t < 0) || (t > 2),
      |         problem = t;
      |         ctr = numios + 1;
      |     end
      | end
      | if problem ~= 0,
      |     error('Type cannot be %i, must be 0, 1 or 2.', problem);
      | end
      mask Callback bin_pts:
      | blk = gcb;
      | mode = get_param(blk, 'mode');
      | current_bins = eval(get_param(blk, 'bin_pts'));
      | if (strcmp(mode, 'one value') || strcmp(mode, 'fields of equal size')) && (length(current_bins) > 1),
      |     error('Only one binary pt may be specified for this mode.');
      | elseif strcmp(mode, 'fields of arbitrary size')
      |     current_names = textscan(strtrim(strrep(strrep(get_param(blk, 'names'), ']', ''), '[', '')), '%s');
      |     current_names = current_names{1};
      |     numios = length(current_names);
      |     if length(current_bins) ~= numios,
      |         error('%d field names specified, but %d binary pts?', numios, length(current_bins));
      |     end
      | end
  vacc_err_cnt1 : Subsystem  Tag=xps:sw_reg  AncestorBlock=xps_library/software register  mask(swreg){mode=one value, io_dir=To Processor, io_delay=1, sample_period=1, names=reg, bitwidths=32, arith_types=0, bin_pts=0, sim_port=off, show_format=off}
      mask prompts: io_dir "I/O direction"; io_delay "I/O delay"; sample_period "Sample period"; names "Name:"; bitwidths "Bitwidth:"; arith_types "Type (ufix=0, fix=1, bool=2):"; bin_pts "Binary pt:"; sim_port "Provide sim input/output?"; show_format "Print format string?"
      mask init:
      | swreg_init(gcb)
      settings: AttributesFormatString=1output
      mask TypeOptions mode: one value | fields of equal size | fields of arbitrary size
      mask Callback mode: swreg_cb(gcb);
      mask TypeOptions io_dir: To Processor | From Processor
      mask Callback io_dir:
      | mask_enables = get_param(gcb, 'MaskEnables');
      | mask_names = get_param(gcb, 'MaskNames');
      | if strcmp(get_param(gcb, 'io_dir'), 'To Processor'),
      |     mask_enables{ismember(mask_names, 'sample_period')} = 'off';
      | else
      |     mask_enables{ismember(mask_names, 'sample_period')} = 'on';
      | end
      | set_param(gcb, 'MaskEnables', mask_enables);
      mask Callback bitwidths:
      | blk = gcb;
      | mode = get_param(blk, 'mode');
      | current_widths = eval(get_param(blk, 'bitwidths'));
      | if (strcmp(mode, 'one value') || strcmp(mode, 'fields of equal size')) && (length(current_widths) > 1),
      |     error('Only one width may be specified for this mode.');
      | elseif strcmp(mode, 'fields of arbitrary size')
      |     current_names = textscan(strtrim(strrep(strrep(get_param(blk, 'names'), ']', ''), '[', '')), '%s');
      |     current_names = current_names{1};
      |     numios = length(current_names);
      |     if length(current_widths) ~= numios,
      |         error('%d field names specified, but %d widths?', numios, length(current_widths));
      |     end
      | end
      | total_width = 0;
      | for ctr = 1 : length(current_widths),
      |     total_width = total_width + current_widths(ctr);
      | end
      | if total_width > 32,
      |     error('Total width must be 32 or less, set to %d.', total_width);
      | end
      mask Callback arith_types:
      | blk = gcb;
      | mode = get_param(blk, 'mode');
      | current_types = eval(get_param(blk, 'arith_types'));
      | numios = length(current_types);
      | if (strcmp(mode, 'one value') || strcmp(mode, 'fields of equal size')) && (length(current_types) > 1),
      |     error('Only one type may be specified for this mode.');
      | elseif strcmp(mode, 'fields of arbitrary size')
      |     current_names = textscan(strtrim(strrep(strrep(get_param(blk, 'names'), ']', ''), '[', '')), '%s');
      |     current_names = current_names{1};
      |     numios = length(current_names);
      |     if length(current_types) ~= numios,
      |         error('%d field names specified, but %d types?', numios, length(current_types));
      |     end
      | end
      | problem = 0;
      | for ctr = 1 : numios,
      |     t = current_types(ctr);
      |     if (t < 0) || (t > 2),
      |         problem = t;
      |         ctr = numios + 1;
      |     end
      | end
      | if problem ~= 0,
      |     error('Type cannot be %i, must be 0, 1 or 2.', problem);
      | end
      mask Callback bin_pts:
      | blk = gcb;
      | mode = get_param(blk, 'mode');
      | current_bins = eval(get_param(blk, 'bin_pts'));
      | if (strcmp(mode, 'one value') || strcmp(mode, 'fields of equal size')) && (length(current_bins) > 1),
      |     error('Only one binary pt may be specified for this mode.');
      | elseif strcmp(mode, 'fields of arbitrary size')
      |     current_names = textscan(strtrim(strrep(strrep(get_param(blk, 'names'), ']', ''), '[', '')), '%s');
      |     current_names = current_names{1};
      |     numios = length(current_names);
      |     if length(current_bins) ~= numios,
      |         error('%d field names specified, but %d binary pts?', numios, length(current_bins));
      |     end
      | end
  vacc_err_cnt2 : Subsystem  Tag=xps:sw_reg  AncestorBlock=xps_library/software register  mask(swreg){mode=one value, io_dir=To Processor, io_delay=1, sample_period=1, names=reg, bitwidths=32, arith_types=0, bin_pts=0, sim_port=off, show_format=off}
      mask prompts: io_dir "I/O direction"; io_delay "I/O delay"; sample_period "Sample period"; names "Name:"; bitwidths "Bitwidth:"; arith_types "Type (ufix=0, fix=1, bool=2):"; bin_pts "Binary pt:"; sim_port "Provide sim input/output?"; show_format "Print format string?"
      mask init:
      | swreg_init(gcb)
      settings: AttributesFormatString=1output
      mask TypeOptions mode: one value | fields of equal size | fields of arbitrary size
      mask Callback mode: swreg_cb(gcb);
      mask TypeOptions io_dir: To Processor | From Processor
      mask Callback io_dir:
      | mask_enables = get_param(gcb, 'MaskEnables');
      | mask_names = get_param(gcb, 'MaskNames');
      | if strcmp(get_param(gcb, 'io_dir'), 'To Processor'),
      |     mask_enables{ismember(mask_names, 'sample_period')} = 'off';
      | else
      |     mask_enables{ismember(mask_names, 'sample_period')} = 'on';
      | end
      | set_param(gcb, 'MaskEnables', mask_enables);
      mask Callback bitwidths:
      | blk = gcb;
      | mode = get_param(blk, 'mode');
      | current_widths = eval(get_param(blk, 'bitwidths'));
      | if (strcmp(mode, 'one value') || strcmp(mode, 'fields of equal size')) && (length(current_widths) > 1),
      |     error('Only one width may be specified for this mode.');
      | elseif strcmp(mode, 'fields of arbitrary size')
      |     current_names = textscan(strtrim(strrep(strrep(get_param(blk, 'names'), ']', ''), '[', '')), '%s');
      |     current_names = current_names{1};
      |     numios = length(current_names);
      |     if length(current_widths) ~= numios,
      |         error('%d field names specified, but %d widths?', numios, length(current_widths));
      |     end
      | end
      | total_width = 0;
      | for ctr = 1 : length(current_widths),
      |     total_width = total_width + current_widths(ctr);
      | end
      | if total_width > 32,
      |     error('Total width must be 32 or less, set to %d.', total_width);
      | end
      mask Callback arith_types:
      | blk = gcb;
      | mode = get_param(blk, 'mode');
      | current_types = eval(get_param(blk, 'arith_types'));
      | numios = length(current_types);
      | if (strcmp(mode, 'one value') || strcmp(mode, 'fields of equal size')) && (length(current_types) > 1),
      |     error('Only one type may be specified for this mode.');
      | elseif strcmp(mode, 'fields of arbitrary size')
      |     current_names = textscan(strtrim(strrep(strrep(get_param(blk, 'names'), ']', ''), '[', '')), '%s');
      |     current_names = current_names{1};
      |     numios = length(current_names);
      |     if length(current_types) ~= numios,
      |         error('%d field names specified, but %d types?', numios, length(current_types));
      |     end
      | end
      | problem = 0;
      | for ctr = 1 : numios,
      |     t = current_types(ctr);
      |     if (t < 0) || (t > 2),
      |         problem = t;
      |         ctr = numios + 1;
      |     end
      | end
      | if problem ~= 0,
      |     error('Type cannot be %i, must be 0, 1 or 2.', problem);
      | end
      mask Callback bin_pts:
      | blk = gcb;
      | mode = get_param(blk, 'mode');
      | current_bins = eval(get_param(blk, 'bin_pts'));
      | if (strcmp(mode, 'one value') || strcmp(mode, 'fields of equal size')) && (length(current_bins) > 1),
      |     error('Only one binary pt may be specified for this mode.');
      | elseif strcmp(mode, 'fields of arbitrary size')
      |     current_names = textscan(strtrim(strrep(strrep(get_param(blk, 'names'), ']', ''), '[', '')), '%s');
      |     current_names = current_names{1};
      |     numios = length(current_names);
      |     if length(current_bins) ~= numios,
      |         error('%d field names specified, but %d binary pts?', numios, length(current_bins));
      |     end
      | end
  vacc_err_cnt3 : Subsystem  Tag=xps:sw_reg  AncestorBlock=xps_library/software register  mask(swreg){mode=one value, io_dir=To Processor, io_delay=1, sample_period=1, names=reg, bitwidths=32, arith_types=0, bin_pts=0, sim_port=off, show_format=off}
      mask prompts: io_dir "I/O direction"; io_delay "I/O delay"; sample_period "Sample period"; names "Name:"; bitwidths "Bitwidth:"; arith_types "Type (ufix=0, fix=1, bool=2):"; bin_pts "Binary pt:"; sim_port "Provide sim input/output?"; show_format "Print format string?"
      mask init:
      | swreg_init(gcb)
      settings: AttributesFormatString=1output
      mask TypeOptions mode: one value | fields of equal size | fields of arbitrary size
      mask Callback mode: swreg_cb(gcb);
      mask TypeOptions io_dir: To Processor | From Processor
      mask Callback io_dir:
      | mask_enables = get_param(gcb, 'MaskEnables');
      | mask_names = get_param(gcb, 'MaskNames');
      | if strcmp(get_param(gcb, 'io_dir'), 'To Processor'),
      |     mask_enables{ismember(mask_names, 'sample_period')} = 'off';
      | else
      |     mask_enables{ismember(mask_names, 'sample_period')} = 'on';
      | end
      | set_param(gcb, 'MaskEnables', mask_enables);
      mask Callback bitwidths:
      | blk = gcb;
      | mode = get_param(blk, 'mode');
      | current_widths = eval(get_param(blk, 'bitwidths'));
      | if (strcmp(mode, 'one value') || strcmp(mode, 'fields of equal size')) && (length(current_widths) > 1),
      |     error('Only one width may be specified for this mode.');
      | elseif strcmp(mode, 'fields of arbitrary size')
      |     current_names = textscan(strtrim(strrep(strrep(get_param(blk, 'names'), ']', ''), '[', '')), '%s');
      |     current_names = current_names{1};
      |     numios = length(current_names);
      |     if length(current_widths) ~= numios,
      |         error('%d field names specified, but %d widths?', numios, length(current_widths));
      |     end
      | end
      | total_width = 0;
      | for ctr = 1 : length(current_widths),
      |     total_width = total_width + current_widths(ctr);
      | end
      | if total_width > 32,
      |     error('Total width must be 32 or less, set to %d.', total_width);
      | end
      mask Callback arith_types:
      | blk = gcb;
      | mode = get_param(blk, 'mode');
      | current_types = eval(get_param(blk, 'arith_types'));
      | numios = length(current_types);
      | if (strcmp(mode, 'one value') || strcmp(mode, 'fields of equal size')) && (length(current_types) > 1),
      |     error('Only one type may be specified for this mode.');
      | elseif strcmp(mode, 'fields of arbitrary size')
      |     current_names = textscan(strtrim(strrep(strrep(get_param(blk, 'names'), ']', ''), '[', '')), '%s');
      |     current_names = current_names{1};
      |     numios = length(current_names);
      |     if length(current_types) ~= numios,
      |         error('%d field names specified, but %d types?', numios, length(current_types));
      |     end
      | end
      | problem = 0;
      | for ctr = 1 : numios,
      |     t = current_types(ctr);
      |     if (t < 0) || (t > 2),
      |         problem = t;
      |         ctr = numios + 1;
      |     end
      | end
      | if problem ~= 0,
      |     error('Type cannot be %i, must be 0, 1 or 2.', problem);
      | end
      mask Callback bin_pts:
      | blk = gcb;
      | mode = get_param(blk, 'mode');
      | current_bins = eval(get_param(blk, 'bin_pts'));
      | if (strcmp(mode, 'one value') || strcmp(mode, 'fields of equal size')) && (length(current_bins) > 1),
      |     error('Only one binary pt may be specified for this mode.');
      | elseif strcmp(mode, 'fields of arbitrary size')
      |     current_names = textscan(strtrim(strrep(strrep(get_param(blk, 'names'), ']', ''), '[', '')), '%s');
      |     current_names = current_names{1};
      |     numios = length(current_names);
      |     if length(current_bins) ~= numios,
      |         error('%d field names specified, but %d binary pts?', numios, length(current_bins));
      |     end
      | end
  vacc_ld_status0 : Subsystem  Tag=xps:sw_reg  AncestorBlock=xps_library/software register  mask(swreg){mode=one value, io_dir=To Processor, io_delay=1, sample_period=1, names=reg, bitwidths=32, arith_types=0, bin_pts=0, sim_port=off, show_format=off}
      mask prompts: io_dir "I/O direction"; io_delay "I/O delay"; sample_period "Sample period"; names "Name:"; bitwidths "Bitwidth:"; arith_types "Type (ufix=0, fix=1, bool=2):"; bin_pts "Binary pt:"; sim_port "Provide sim input/output?"; show_format "Print format string?"
      mask init:
      | swreg_init(gcb)
      settings: AttributesFormatString=1output
      mask TypeOptions mode: one value | fields of equal size | fields of arbitrary size
      mask Callback mode: swreg_cb(gcb);
      mask TypeOptions io_dir: To Processor | From Processor
      mask Callback io_dir:
      | mask_enables = get_param(gcb, 'MaskEnables');
      | mask_names = get_param(gcb, 'MaskNames');
      | if strcmp(get_param(gcb, 'io_dir'), 'To Processor'),
      |     mask_enables{ismember(mask_names, 'sample_period')} = 'off';
      | else
      |     mask_enables{ismember(mask_names, 'sample_period')} = 'on';
      | end
      | set_param(gcb, 'MaskEnables', mask_enables);
      mask Callback bitwidths:
      | blk = gcb;
      | mode = get_param(blk, 'mode');
      | current_widths = eval(get_param(blk, 'bitwidths'));
      | if (strcmp(mode, 'one value') || strcmp(mode, 'fields of equal size')) && (length(current_widths) > 1),
      |     error('Only one width may be specified for this mode.');
      | elseif strcmp(mode, 'fields of arbitrary size')
      |     current_names = textscan(strtrim(strrep(strrep(get_param(blk, 'names'), ']', ''), '[', '')), '%s');
      |     current_names = current_names{1};
      |     numios = length(current_names);
      |     if length(current_widths) ~= numios,
      |         error('%d field names specified, but %d widths?', numios, length(current_widths));
      |     end
      | end
      | total_width = 0;
      | for ctr = 1 : length(current_widths),
      |     total_width = total_width + current_widths(ctr);
      | end
      | if total_width > 32,
      |     error('Total width must be 32 or less, set to %d.', total_width);
      | end
      mask Callback arith_types:
      | blk = gcb;
      | mode = get_param(blk, 'mode');
      | current_types = eval(get_param(blk, 'arith_types'));
      | numios = length(current_types);
      | if (strcmp(mode, 'one value') || strcmp(mode, 'fields of equal size')) && (length(current_types) > 1),
      |     error('Only one type may be specified for this mode.');
      | elseif strcmp(mode, 'fields of arbitrary size')
      |     current_names = textscan(strtrim(strrep(strrep(get_param(blk, 'names'), ']', ''), '[', '')), '%s');
      |     current_names = current_names{1};
      |     numios = length(current_names);
      |     if length(current_types) ~= numios,
      |         error('%d field names specified, but %d types?', numios, length(current_types));
      |     end
      | end
      | problem = 0;
      | for ctr = 1 : numios,
      |     t = current_types(ctr);
      |     if (t < 0) || (t > 2),
      |         problem = t;
      |         ctr = numios + 1;
      |     end
      | end
      | if problem ~= 0,
      |     error('Type cannot be %i, must be 0, 1 or 2.', problem);
      | end
      mask Callback bin_pts:
      | blk = gcb;
      | mode = get_param(blk, 'mode');
      | current_bins = eval(get_param(blk, 'bin_pts'));
      | if (strcmp(mode, 'one value') || strcmp(mode, 'fields of equal size')) && (length(current_bins) > 1),
      |     error('Only one binary pt may be specified for this mode.');
      | elseif strcmp(mode, 'fields of arbitrary size')
      |     current_names = textscan(strtrim(strrep(strrep(get_param(blk, 'names'), ']', ''), '[', '')), '%s');
      |     current_names = current_names{1};
      |     numios = length(current_names);
      |     if length(current_bins) ~= numios,
      |         error('%d field names specified, but %d binary pts?', numios, length(current_bins));
      |     end
      | end
  vacc_ld_status1 : Subsystem  Tag=xps:sw_reg  AncestorBlock=xps_library/software register  mask(swreg){mode=one value, io_dir=To Processor, io_delay=1, sample_period=1, names=reg, bitwidths=32, arith_types=0, bin_pts=0, sim_port=off, show_format=off}
      mask prompts: io_dir "I/O direction"; io_delay "I/O delay"; sample_period "Sample period"; names "Name:"; bitwidths "Bitwidth:"; arith_types "Type (ufix=0, fix=1, bool=2):"; bin_pts "Binary pt:"; sim_port "Provide sim input/output?"; show_format "Print format string?"
      mask init:
      | swreg_init(gcb)
      settings: AttributesFormatString=1output
      mask TypeOptions mode: one value | fields of equal size | fields of arbitrary size
      mask Callback mode: swreg_cb(gcb);
      mask TypeOptions io_dir: To Processor | From Processor
      mask Callback io_dir:
      | mask_enables = get_param(gcb, 'MaskEnables');
      | mask_names = get_param(gcb, 'MaskNames');
      | if strcmp(get_param(gcb, 'io_dir'), 'To Processor'),
      |     mask_enables{ismember(mask_names, 'sample_period')} = 'off';
      | else
      |     mask_enables{ismember(mask_names, 'sample_period')} = 'on';
      | end
      | set_param(gcb, 'MaskEnables', mask_enables);
      mask Callback bitwidths:
      | blk = gcb;
      | mode = get_param(blk, 'mode');
      | current_widths = eval(get_param(blk, 'bitwidths'));
      | if (strcmp(mode, 'one value') || strcmp(mode, 'fields of equal size')) && (length(current_widths) > 1),
      |     error('Only one width may be specified for this mode.');
      | elseif strcmp(mode, 'fields of arbitrary size')
      |     current_names = textscan(strtrim(strrep(strrep(get_param(blk, 'names'), ']', ''), '[', '')), '%s');
      |     current_names = current_names{1};
      |     numios = length(current_names);
      |     if length(current_widths) ~= numios,
      |         error('%d field names specified, but %d widths?', numios, length(current_widths));
      |     end
      | end
      | total_width = 0;
      | for ctr = 1 : length(current_widths),
      |     total_width = total_width + current_widths(ctr);
      | end
      | if total_width > 32,
      |     error('Total width must be 32 or less, set to %d.', total_width);
      | end
      mask Callback arith_types:
      | blk = gcb;
      | mode = get_param(blk, 'mode');
      | current_types = eval(get_param(blk, 'arith_types'));
      | numios = length(current_types);
      | if (strcmp(mode, 'one value') || strcmp(mode, 'fields of equal size')) && (length(current_types) > 1),
      |     error('Only one type may be specified for this mode.');
      | elseif strcmp(mode, 'fields of arbitrary size')
      |     current_names = textscan(strtrim(strrep(strrep(get_param(blk, 'names'), ']', ''), '[', '')), '%s');
      |     current_names = current_names{1};
      |     numios = length(current_names);
      |     if length(current_types) ~= numios,
      |         error('%d field names specified, but %d types?', numios, length(current_types));
      |     end
      | end
      | problem = 0;
      | for ctr = 1 : numios,
      |     t = current_types(ctr);
      |     if (t < 0) || (t > 2),
      |         problem = t;
      |         ctr = numios + 1;
      |     end
      | end
      | if problem ~= 0,
      |     error('Type cannot be %i, must be 0, 1 or 2.', problem);
      | end
      mask Callback bin_pts:
      | blk = gcb;
      | mode = get_param(blk, 'mode');
      | current_bins = eval(get_param(blk, 'bin_pts'));
      | if (strcmp(mode, 'one value') || strcmp(mode, 'fields of equal size')) && (length(current_bins) > 1),
      |     error('Only one binary pt may be specified for this mode.');
      | elseif strcmp(mode, 'fields of arbitrary size')
      |     current_names = textscan(strtrim(strrep(strrep(get_param(blk, 'names'), ']', ''), '[', '')), '%s');
      |     current_names = current_names{1};
      |     numios = length(current_names);
      |     if length(current_bins) ~= numios,
      |         error('%d field names specified, but %d binary pts?', numios, length(current_bins));
      |     end
      | end
  vacc_ld_status2 : Subsystem  Tag=xps:sw_reg  AncestorBlock=xps_library/software register  mask(swreg){mode=one value, io_dir=To Processor, io_delay=1, sample_period=1, names=reg, bitwidths=32, arith_types=0, bin_pts=0, sim_port=off, show_format=off}
      mask prompts: io_dir "I/O direction"; io_delay "I/O delay"; sample_period "Sample period"; names "Name:"; bitwidths "Bitwidth:"; arith_types "Type (ufix=0, fix=1, bool=2):"; bin_pts "Binary pt:"; sim_port "Provide sim input/output?"; show_format "Print format string?"
      mask init:
      | swreg_init(gcb)
      settings: AttributesFormatString=1output
      mask TypeOptions mode: one value | fields of equal size | fields of arbitrary size
      mask Callback mode: swreg_cb(gcb);
      mask TypeOptions io_dir: To Processor | From Processor
      mask Callback io_dir:
      | mask_enables = get_param(gcb, 'MaskEnables');
      | mask_names = get_param(gcb, 'MaskNames');
      | if strcmp(get_param(gcb, 'io_dir'), 'To Processor'),
      |     mask_enables{ismember(mask_names, 'sample_period')} = 'off';
      | else
      |     mask_enables{ismember(mask_names, 'sample_period')} = 'on';
      | end
      | set_param(gcb, 'MaskEnables', mask_enables);
      mask Callback bitwidths:
      | blk = gcb;
      | mode = get_param(blk, 'mode');
      | current_widths = eval(get_param(blk, 'bitwidths'));
      | if (strcmp(mode, 'one value') || strcmp(mode, 'fields of equal size')) && (length(current_widths) > 1),
      |     error('Only one width may be specified for this mode.');
      | elseif strcmp(mode, 'fields of arbitrary size')
      |     current_names = textscan(strtrim(strrep(strrep(get_param(blk, 'names'), ']', ''), '[', '')), '%s');
      |     current_names = current_names{1};
      |     numios = length(current_names);
      |     if length(current_widths) ~= numios,
      |         error('%d field names specified, but %d widths?', numios, length(current_widths));
      |     end
      | end
      | total_width = 0;
      | for ctr = 1 : length(current_widths),
      |     total_width = total_width + current_widths(ctr);
      | end
      | if total_width > 32,
      |     error('Total width must be 32 or less, set to %d.', total_width);
      | end
      mask Callback arith_types:
      | blk = gcb;
      | mode = get_param(blk, 'mode');
      | current_types = eval(get_param(blk, 'arith_types'));
      | numios = length(current_types);
      | if (strcmp(mode, 'one value') || strcmp(mode, 'fields of equal size')) && (length(current_types) > 1),
      |     error('Only one type may be specified for this mode.');
      | elseif strcmp(mode, 'fields of arbitrary size')
      |     current_names = textscan(strtrim(strrep(strrep(get_param(blk, 'names'), ']', ''), '[', '')), '%s');
      |     current_names = current_names{1};
      |     numios = length(current_names);
      |     if length(current_types) ~= numios,
      |         error('%d field names specified, but %d types?', numios, length(current_types));
      |     end
      | end
      | problem = 0;
      | for ctr = 1 : numios,
      |     t = current_types(ctr);
      |     if (t < 0) || (t > 2),
      |         problem = t;
      |         ctr = numios + 1;
      |     end
      | end
      | if problem ~= 0,
      |     error('Type cannot be %i, must be 0, 1 or 2.', problem);
      | end
      mask Callback bin_pts:
      | blk = gcb;
      | mode = get_param(blk, 'mode');
      | current_bins = eval(get_param(blk, 'bin_pts'));
      | if (strcmp(mode, 'one value') || strcmp(mode, 'fields of equal size')) && (length(current_bins) > 1),
      |     error('Only one binary pt may be specified for this mode.');
      | elseif strcmp(mode, 'fields of arbitrary size')
      |     current_names = textscan(strtrim(strrep(strrep(get_param(blk, 'names'), ']', ''), '[', '')), '%s');
      |     current_names = current_names{1};
      |     numios = length(current_names);
      |     if length(current_bins) ~= numios,
      |         error('%d field names specified, but %d binary pts?', numios, length(current_bins));
      |     end
      | end
  vacc_ld_status3 : Subsystem  Tag=xps:sw_reg  AncestorBlock=xps_library/software register  mask(swreg){mode=one value, io_dir=To Processor, io_delay=1, sample_period=1, names=reg, bitwidths=32, arith_types=0, bin_pts=0, sim_port=off, show_format=off}
      mask prompts: io_dir "I/O direction"; io_delay "I/O delay"; sample_period "Sample period"; names "Name:"; bitwidths "Bitwidth:"; arith_types "Type (ufix=0, fix=1, bool=2):"; bin_pts "Binary pt:"; sim_port "Provide sim input/output?"; show_format "Print format string?"
      mask init:
      | swreg_init(gcb)
      settings: AttributesFormatString=1output
      mask TypeOptions mode: one value | fields of equal size | fields of arbitrary size
      mask Callback mode: swreg_cb(gcb);
      mask TypeOptions io_dir: To Processor | From Processor
      mask Callback io_dir:
      | mask_enables = get_param(gcb, 'MaskEnables');
      | mask_names = get_param(gcb, 'MaskNames');
      | if strcmp(get_param(gcb, 'io_dir'), 'To Processor'),
      |     mask_enables{ismember(mask_names, 'sample_period')} = 'off';
      | else
      |     mask_enables{ismember(mask_names, 'sample_period')} = 'on';
      | end
      | set_param(gcb, 'MaskEnables', mask_enables);
      mask Callback bitwidths:
      | blk = gcb;
      | mode = get_param(blk, 'mode');
      | current_widths = eval(get_param(blk, 'bitwidths'));
      | if (strcmp(mode, 'one value') || strcmp(mode, 'fields of equal size')) && (length(current_widths) > 1),
      |     error('Only one width may be specified for this mode.');
      | elseif strcmp(mode, 'fields of arbitrary size')
      |     current_names = textscan(strtrim(strrep(strrep(get_param(blk, 'names'), ']', ''), '[', '')), '%s');
      |     current_names = current_names{1};
      |     numios = length(current_names);
      |     if length(current_widths) ~= numios,
      |         error('%d field names specified, but %d widths?', numios, length(current_widths));
      |     end
      | end
      | total_width = 0;
      | for ctr = 1 : length(current_widths),
      |     total_width = total_width + current_widths(ctr);
      | end
      | if total_width > 32,
      |     error('Total width must be 32 or less, set to %d.', total_width);
      | end
      mask Callback arith_types:
      | blk = gcb;
      | mode = get_param(blk, 'mode');
      | current_types = eval(get_param(blk, 'arith_types'));
      | numios = length(current_types);
      | if (strcmp(mode, 'one value') || strcmp(mode, 'fields of equal size')) && (length(current_types) > 1),
      |     error('Only one type may be specified for this mode.');
      | elseif strcmp(mode, 'fields of arbitrary size')
      |     current_names = textscan(strtrim(strrep(strrep(get_param(blk, 'names'), ']', ''), '[', '')), '%s');
      |     current_names = current_names{1};
      |     numios = length(current_names);
      |     if length(current_types) ~= numios,
      |         error('%d field names specified, but %d types?', numios, length(current_types));
      |     end
      | end
      | problem = 0;
      | for ctr = 1 : numios,
      |     t = current_types(ctr);
      |     if (t < 0) || (t > 2),
      |         problem = t;
      |         ctr = numios + 1;
      |     end
      | end
      | if problem ~= 0,
      |     error('Type cannot be %i, must be 0, 1 or 2.', problem);
      | end
      mask Callback bin_pts:
      | blk = gcb;
      | mode = get_param(blk, 'mode');
      | current_bins = eval(get_param(blk, 'bin_pts'));
      | if (strcmp(mode, 'one value') || strcmp(mode, 'fields of equal size')) && (length(current_bins) > 1),
      |     error('Only one binary pt may be specified for this mode.');
      | elseif strcmp(mode, 'fields of arbitrary size')
      |     current_names = textscan(strtrim(strrep(strrep(get_param(blk, 'names'), ']', ''), '[', '')), '%s');
      |     current_names = current_names{1};
      |     numios = length(current_names);
      |     if length(current_bins) ~= numios,
      |         error('%d field names specified, but %d binary pts?', numios, length(current_bins));
      |     end
      | end
  vacc_monitor : Subsystem
  vacc_monitor1 : Subsystem
  vacc_monitor2 : Subsystem
  vacc_monitor3 : Subsystem
  vacc_monitor4 : Subsystem
  vacc_monitor5 : Subsystem
  vacc_monitor6 : Subsystem
  vacc_monitor7 : Subsystem
  vacc_time_lsw : Subsystem  Tag=xps:sw_reg  AncestorBlock=xps_library/software register  mask(swreg){mode=one value, io_dir=From Processor, io_delay=1, sample_period=1, names=reg, bitwidths=32, arith_types=0, bin_pts=0, sim_port=on, show_format=off}
      mask prompts: io_dir "I/O direction"; io_delay "I/O delay"; sample_period "Sample period"; names "Name:"; bitwidths "Bitwidth:"; arith_types "Type (ufix=0, fix=1, bool=2):"; bin_pts "Binary pt:"; sim_port "Provide sim input/output?"; show_format "Print format string?"
      mask init:
      | swreg_init(gcb)
      settings: AttributesFormatString=1input
      mask TypeOptions mode: one value | fields of equal size | fields of arbitrary size
      mask Callback mode: swreg_cb(gcb);
      mask TypeOptions io_dir: To Processor | From Processor
      mask Callback io_dir:
      | mask_enables = get_param(gcb, 'MaskEnables');
      | mask_names = get_param(gcb, 'MaskNames');
      | if strcmp(get_param(gcb, 'io_dir'), 'To Processor'),
      |     mask_enables{ismember(mask_names, 'sample_period')} = 'off';
      | else
      |     mask_enables{ismember(mask_names, 'sample_period')} = 'on';
      | end
      | set_param(gcb, 'MaskEnables', mask_enables);
      mask Callback bitwidths:
      | blk = gcb;
      | mode = get_param(blk, 'mode');
      | current_widths = eval(get_param(blk, 'bitwidths'));
      | if (strcmp(mode, 'one value') || strcmp(mode, 'fields of equal size')) && (length(current_widths) > 1),
      |     error('Only one width may be specified for this mode.');
      | elseif strcmp(mode, 'fields of arbitrary size')
      |     current_names = textscan(strtrim(strrep(strrep(get_param(blk, 'names'), ']', ''), '[', '')), '%s');
      |     current_names = current_names{1};
      |     numios = length(current_names);
      |     if length(current_widths) ~= numios,
      |         error('%d field names specified, but %d widths?', numios, length(current_widths));
      |     end
      | end
      | total_width = 0;
      | for ctr = 1 : length(current_widths),
      |     total_width = total_width + current_widths(ctr);
      | end
      | if total_width > 32,
      |     error('Total width must be 32 or less, set to %d.', total_width);
      | end
      mask Callback arith_types:
      | blk = gcb;
      | mode = get_param(blk, 'mode');
      | current_types = eval(get_param(blk, 'arith_types'));
      | numios = length(current_types);
      | if (strcmp(mode, 'one value') || strcmp(mode, 'fields of equal size')) && (length(current_types) > 1),
      |     error('Only one type may be specified for this mode.');
      | elseif strcmp(mode, 'fields of arbitrary size')
      |     current_names = textscan(strtrim(strrep(strrep(get_param(blk, 'names'), ']', ''), '[', '')), '%s');
      |     current_names = current_names{1};
      |     numios = length(current_names);
      |     if length(current_types) ~= numios,
      |         error('%d field names specified, but %d types?', numios, length(current_types));
      |     end
      | end
      | problem = 0;
      | for ctr = 1 : numios,
      |     t = current_types(ctr);
      |     if (t < 0) || (t > 2),
      |         problem = t;
      |         ctr = numios + 1;
      |     end
      | end
      | if problem ~= 0,
      |     error('Type cannot be %i, must be 0, 1 or 2.', problem);
      | end
      mask Callback bin_pts:
      | blk = gcb;
      | mode = get_param(blk, 'mode');
      | current_bins = eval(get_param(blk, 'bin_pts'));
      | if (strcmp(mode, 'one value') || strcmp(mode, 'fields of equal size')) && (length(current_bins) > 1),
      |     error('Only one binary pt may be specified for this mode.');
      | elseif strcmp(mode, 'fields of arbitrary size')
      |     current_names = textscan(strtrim(strrep(strrep(get_param(blk, 'names'), ']', ''), '[', '')), '%s');
      |     current_names = current_names{1};
      |     numios = length(current_names);
      |     if length(current_bins) ~= numios,
      |         error('%d field names specified, but %d binary pts?', numios, length(current_bins));
      |     end
      | end
  vacc_time_msw : Subsystem  Tag=xps:sw_reg  AncestorBlock=xps_library/software register  mask(swreg){mode=fields of arbitrary size, io_dir=From Processor, io_delay=1, sample_period=1, names=[arm msw], bitwidths=[1 16], arith_types=[2 0], bin_pts=[0 0], sim_port=off, show_format=off}
      mask prompts: io_dir "I/O direction"; io_delay "I/O delay"; sample_period "Sample period"; names "Names [msb ... lsb]:"; bitwidths "Bitwidths [msb ... lsb]:"; arith_types "Types (ufix=0, fix=1, bool=2) [msb ... lsb]:"; bin_pts "Binary pts [msb ... lsb]:"; sim_port "Provide sim input/output?"; show_format "Print format string?"
      mask init:
      | swreg_init(gcb)
      settings: AttributesFormatString=2 inputs
      mask TypeOptions mode: one value | fields of equal size | fields of arbitrary size
      mask Callback mode: swreg_cb(gcb);
      mask TypeOptions io_dir: To Processor | From Processor
      mask Callback io_dir:
      | mask_enables = get_param(gcb, 'MaskEnables');
      | mask_names = get_param(gcb, 'MaskNames');
      | if strcmp(get_param(gcb, 'io_dir'), 'To Processor'),
      |     mask_enables{ismember(mask_names, 'sample_period')} = 'off';
      | else
      |     mask_enables{ismember(mask_names, 'sample_period')} = 'on';
      | end
      | set_param(gcb, 'MaskEnables', mask_enables);
      mask Callback bitwidths:
      | blk = gcb;
      | mode = get_param(blk, 'mode');
      | current_widths = eval(get_param(blk, 'bitwidths'));
      | if (strcmp(mode, 'one value') || strcmp(mode, 'fields of equal size')) && (length(current_widths) > 1),
      |     error('Only one width may be specified for this mode.');
      | elseif strcmp(mode, 'fields of arbitrary size')
      |     current_names = textscan(strtrim(strrep(strrep(get_param(blk, 'names'), ']', ''), '[', '')), '%s');
      |     current_names = current_names{1};
      |     numios = length(current_names);
      |     if length(current_widths) ~= numios,
      |         error('%d field names specified, but %d widths?', numios, length(current_widths));
      |     end
      | end
      | total_width = 0;
      | for ctr = 1 : length(current_widths),
      |     total_width = total_width + current_widths(ctr);
      | end
      | if total_width > 32,
      |     error('Total width must be 32 or less, set to %d.', total_width);
      | end
      mask Callback arith_types:
      | blk = gcb;
      | mode = get_param(blk, 'mode');
      | current_types = eval(get_param(blk, 'arith_types'));
      | numios = length(current_types);
      | if (strcmp(mode, 'one value') || strcmp(mode, 'fields of equal size')) && (length(current_types) > 1),
      |     error('Only one type may be specified for this mode.');
      | elseif strcmp(mode, 'fields of arbitrary size')
      |     current_names = textscan(strtrim(strrep(strrep(get_param(blk, 'names'), ']', ''), '[', '')), '%s');
      |     current_names = current_names{1};
      |     numios = length(current_names);
      |     if length(current_types) ~= numios,
      |         error('%d field names specified, but %d types?', numios, length(current_types));
      |     end
      | end
      | problem = 0;
      | for ctr = 1 : numios,
      |     t = current_types(ctr);
      |     if (t < 0) || (t > 2),
      |         problem = t;
      |         ctr = numios + 1;
      |     end
      | end
      | if problem ~= 0,
      |     error('Type cannot be %i, must be 0, 1 or 2.', problem);
      | end
      mask Callback bin_pts:
      | blk = gcb;
      | mode = get_param(blk, 'mode');
      | current_bins = eval(get_param(blk, 'bin_pts'));
      | if (strcmp(mode, 'one value') || strcmp(mode, 'fields of equal size')) && (length(current_bins) > 1),
      |     error('Only one binary pt may be specified for this mode.');
      | elseif strcmp(mode, 'fields of arbitrary size')
      |     current_names = textscan(strtrim(strrep(strrep(get_param(blk, 'names'), ']', ''), '[', '')), '%s');
      |     current_names = current_names{1};
      |     numios = length(current_names);
      |     if length(current_bins) ~= numios,
      |         error('%d field names specified, but %d binary pts?', numios, length(current_bins));
      |     end
      | end
  vacc_tvg0 : Subsystem  AncestorBlock=casper_library/Accumulators/vacc_tvg  mask{len=(4*(4+1))/2*8*2^(12-5)}
      mask prompts: len "Number of Vectors"
      mask init:
      | fmtstr = sprintf('Vector Length: %d', len);
      | set_param(gcb, 'AttributesFormatString', fmtstr);
      settings: AttributesFormatString=Vector Length: 10240
  vacc_tvg1 : Subsystem  AncestorBlock=casper_library/Accumulators/vacc_tvg  mask{len=(4*(4+1))/2*8*2^(12-5)}
      mask prompts: len "Number of Vectors"
      mask init:
      | fmtstr = sprintf('Vector Length: %d', len);
      | set_param(gcb, 'AttributesFormatString', fmtstr);
      settings: AttributesFormatString=Vector Length: 10240
  vacc_tvg2 : Subsystem  AncestorBlock=casper_library/Accumulators/vacc_tvg  mask{len=(4*(4+1))/2*8*2^(12-5)}
      mask prompts: len "Number of Vectors"
      mask init:
      | fmtstr = sprintf('Vector Length: %d', len);
      | set_param(gcb, 'AttributesFormatString', fmtstr);
      settings: AttributesFormatString=Vector Length: 10240
  vacc_tvg3 : Subsystem  AncestorBlock=casper_library/Accumulators/vacc_tvg  mask{len=(4*(4+1))/2*8*2^(12-5)}
      mask prompts: len "Number of Vectors"
      mask init:
      | fmtstr = sprintf('Vector Length: %d', len);
      | set_param(gcb, 'AttributesFormatString', fmtstr);
      settings: AttributesFormatString=Vector Length: 10240
  xeng0 : Subsystem  Tag=casper:xeng  AncestorBlock=casper_library_correlator/xeng  mask(xeng){n_ants=4, n_bits=8, acc_len=256, demux_factor=8, add_latency=2, mult_latency=4, bram_latency=6, use_ded_mult=1, use_bram_delay=1}
      mask prompts: n_ants "Number of antennas"; n_bits "Bit-width of samples in"; acc_len "Accumulation length"; add_latency "Adder latency"; mult_latency "Multiplier latency"; bram_latency "BRAM latency"; use_ded_mult "Implementation: Multiplier type (0=slices 1=embedded 2=bram)"; use_bram_delay "Implementation: Delay type (0=SLR, 1=BRAM)"
      mask help: CASPER X engine with added internal valid data masking functionality, descramble and integral demux. Based on Aaron Parsons' and Lynn Urry's original X engine design.
      mask init:
      | xeng_init(gcb, ...
      |     'n_ants', n_ants, ...
      |     'n_bits', n_bits, ...
      |     'acc_len', acc_len, ...
      |     'demux_factor', demux_factor, ...
      |     'add_latency', add_latency, ...
      |     'mult_latency', mult_latency, ...
      |     'bram_latency', bram_latency, ...
      |     'use_ded_mult', use_ded_mult, ...
      |     'use_bram_delay', use_bram_delay);
      settings: AttributesFormatString=n_ant=4, bits=8, mult_typ=1, bram_typ=1
      mask TypeOptions demux_factor: 1 | 2 | 4 | 8
  xeng1 : Subsystem  Tag=casper:xeng  AncestorBlock=casper_library_correlator/xeng  mask(xeng){n_ants=4, n_bits=8, acc_len=256, demux_factor=8, add_latency=2, mult_latency=4, bram_latency=6, use_ded_mult=1, use_bram_delay=1}
      mask prompts: n_ants "Number of antennas"; n_bits "Bit-width of samples in"; acc_len "Accumulation length"; add_latency "Adder latency"; mult_latency "Multiplier latency"; bram_latency "BRAM latency"; use_ded_mult "Implementation: Multiplier type (0=slices 1=embedded 2=bram)"; use_bram_delay "Implementation: Delay type (0=SLR, 1=BRAM)"
      mask help: CASPER X engine with added internal valid data masking functionality, descramble and integral demux. Based on Aaron Parsons' and Lynn Urry's original X engine design.
      mask init: same as r2_2f_4x_4a_4k_r366/xeng0
      settings: AttributesFormatString=n_ant=4, bits=8, mult_typ=1, bram_typ=1
      mask TypeOptions demux_factor: 1 | 2 | 4 | 8
  xeng2 : Subsystem  Tag=casper:xeng  AncestorBlock=casper_library_correlator/xeng  mask(xeng){n_ants=4, n_bits=8, acc_len=256, demux_factor=8, add_latency=2, mult_latency=4, bram_latency=6, use_ded_mult=1, use_bram_delay=1}
      mask prompts: n_ants "Number of antennas"; n_bits "Bit-width of samples in"; acc_len "Accumulation length"; add_latency "Adder latency"; mult_latency "Multiplier latency"; bram_latency "BRAM latency"; use_ded_mult "Implementation: Multiplier type (0=slices 1=embedded 2=bram)"; use_bram_delay "Implementation: Delay type (0=SLR, 1=BRAM)"
      mask help: CASPER X engine with added internal valid data masking functionality, descramble and integral demux. Based on Aaron Parsons' and Lynn Urry's original X engine design.
      mask init: same as r2_2f_4x_4a_4k_r366/xeng0
      settings: AttributesFormatString=n_ant=4, bits=8, mult_typ=1, bram_typ=1
      mask TypeOptions demux_factor: 1 | 2 | 4 | 8
  xeng3 : Subsystem  Tag=casper:xeng  AncestorBlock=casper_library_correlator/xeng  mask(xeng){n_ants=4, n_bits=8, acc_len=256, demux_factor=8, add_latency=2, mult_latency=4, bram_latency=6, use_ded_mult=1, use_bram_delay=1}
      mask prompts: n_ants "Number of antennas"; n_bits "Bit-width of samples in"; acc_len "Accumulation length"; add_latency "Adder latency"; mult_latency "Multiplier latency"; bram_latency "BRAM latency"; use_ded_mult "Implementation: Multiplier type (0=slices 1=embedded 2=bram)"; use_bram_delay "Implementation: Delay type (0=SLR, 1=BRAM)"
      mask help: CASPER X engine with added internal valid data masking functionality, descramble and integral demux. Based on Aaron Parsons' and Lynn Urry's original X engine design.
      mask init: same as r2_2f_4x_4a_4k_r366/xeng0
      settings: AttributesFormatString=n_ant=4, bits=8, mult_typ=1, bram_typ=1
      mask TypeOptions demux_factor: 1 | 2 | 4 | 8
  xeng_tvg0 : Subsystem  AncestorBlock=casper_library/Correlator/xeng_tvg  mask{ant_bits=2, x_int_bits=8, sync_period=16}
      mask prompts: ant_bits "Number of Antennas (2^?):"; x_int_bits "X Integration Length (2^?):"; sync_period "Sync Pulse Period (2^?):"
  xeng_tvg1 : Subsystem  AncestorBlock=casper_library/Correlator/xeng_tvg  mask{ant_bits=2, x_int_bits=8, sync_period=16}
      mask prompts: ant_bits "Number of Antennas (2^?):"; x_int_bits "X Integration Length (2^?):"; sync_period "Sync Pulse Period (2^?):"
  xeng_tvg2 : Subsystem  AncestorBlock=casper_library/Correlator/xeng_tvg  mask{ant_bits=2, x_int_bits=8, sync_period=16}
      mask prompts: ant_bits "Number of Antennas (2^?):"; x_int_bits "X Integration Length (2^?):"; sync_period "Sync Pulse Period (2^?):"
  xeng_tvg3 : Subsystem  AncestorBlock=casper_library/Correlator/xeng_tvg  mask{ant_bits=2, x_int_bits=8, sync_period=16}
      mask prompts: ant_bits "Number of Antennas (2^?):"; x_int_bits "X Integration Length (2^?):"; sync_period "Sync Pulse Period (2^?):"
  wires:
  master_reset_sim4/1 -> acc_len/1(sim_1)
  acc_len/1(in_reg) -> [acc_len]
  err_clear_sim2/1 -> Subsystem2/5(data_sel)
  err_clear_sim6/1 -> Subsystem2/4(valid_sel)
  err_clear_sim7/1 -> Subsystem2/3(inj_vector)
  err_clear_sim8/1 -> Subsystem2/2(inj_counter)
  Pulse Generator1/1 -> Subsystem2/1(new_acc)
  err_clear_sim9/1 -> Subsystem2/6(run)
  Subsystem2/1(Out1) -> Terminator37/1
  Delay17/1(q) -> negedge_delay/1(in)
  xeng_tvg0/1(sync_out) -> Delay56/1(d)
  xeng_tvg0/2(data_out) -> Delay73/1(d)
  xeng_tvg0/3(valid_out) -> Delay74/1(d)
  xeng0/1(sync_out) -> Delay30/1(d)
  xeng0/2(acc) -> Delay31/1(d)
  xeng0/3(valid) -> Delay45/1(d)
  [vacc_tvg_sel] -> vacc_tvg0/1(tvg_sel)
  Delay151/1(q) -> Delay83/1(d)
  Delay118/1(q) -> negedge_delay1/1(in)
  16b_32b/1(Out1) -> snap_xeng0/1(din), vacc_tvg0/3(data_in)
  vacc_tvg0/1(sync_out) -> fake_vacc0/5(sync_in)
  vacc_tvg0/2(data_out) -> fake_vacc0/6(data_in)
  vacc_tvg0/3(valid_out) -> fake_vacc0/7(we)
  [acc_len] -> fake_vacc0/4(acc_len)
  xeng0/4(mcnt_out) -> Delay46/1(d)
  vacc_monitor/2(spec_cnt) -> vacc_cnt0/1(out_reg)
  vacc_monitor/1(error_cnt) -> vacc_err_cnt0/1(out_reg)
  fake_vacc0/1(new_acc) -> [new_acc0]
  [cnt_rst] -> vacc_monitor/1(cnt_rst)
  fake_vacc0/7(timestamp) -> delay7/1
  Delay56/1(q) -> xeng0/1(sync_in)
  Delay73/1(q) -> xeng0/2(ant)
  Delay74/1(q) -> xeng0/3(window_valid)
  Delay83/1(q) -> xeng0/4(mcnt_in)
  [vacc_ld_arm] -> fake_vacc0/2(arm)
  [vacc_ld_time] -> fake_vacc0/3(load_time)
  [vacc_rst] -> fake_vacc0/1(rst)
  delay5/1 -> fake_vacc0/8(pcnt_in)
  fake_vacc0/10(error_out) -> [vacc_err0]
  [new_acc0] -> vacc_monitor/2(new_acc)
  [vacc_err0] -> vacc_monitor/3(error)
  Delay27/1(q) -> negedge_delay2/1(in)
  Delay96/1(q) -> negedge_delay3/1(in)
  Delay97/1(q) -> negedge_delay4/1(in)
  fake_vacc0/2(data_out) -> delay4/1
  fake_vacc0/4(valid_out) -> delay2/1
  fake_vacc0/6(rb_done) -> delay6/1
  [vacc_ld_stat0] -> vacc_ld_status0/1(out_reg)
  fake_vacc0/8(ld_status) -> [vacc_ld_stat0]
  [id0] -> pack_out0/6(xeng_id)
  [vacc_err0] -> snap_vacc0/4(stop)
  pack_out0/3(eof) -> Delay15/1(d)
  [cnt_rst] -> vacc_monitor2/1(cnt_rst)
  vacc_monitor2/1(pkt_cnt) -> pack_out_cnt0/1(out_reg)
  vacc_monitor2/2(error_cnt) -> pack_out_err0/1(out_reg)
  pack_out0/5(fetch) -> fake_vacc0/9(re)
  delay4/1 -> snap_vacc0/1(din), pack_out0/1(data_in)
  delay2/1 -> snap_vacc0/2(we), pack_out0/2(valid_in)
  delay6/1 -> snap_vacc0/3(trig), pack_out0/4(rb_done)
  delay7/1 -> pack_out0/5(timestamp)
  pack_out0/1(data_out) -> Delay23/1(d)
  pack_out0/4(err) -> Delay34/1(d)
  Delay34/1(q) -> [pack_err0], vacc_monitor2/3(error)
  negedge_delay3/1(out) -> front_panel/6(led2_red)
  negedge_delay4/1(out) -> front_panel/7(led3_red)
  [flasher_en] -> front_panel/1(flasher_en)
  [new_acc0] -> front_panel/2(sync)
  [xsync_out0] -> front_panel/3(step)
  negedge_delay2/1(out) -> front_panel/4(led0_red)
  negedge_delay/1(out) -> front_panel/10(led6_green)
  negedge_delay1/1(out) -> front_panel/9(led5_green)
  txport/1(in_txport) -> Delay9/1(d)
  txip/1(in_txip) -> Delay10/1(d)
  Delay9/1(q) -> [gbe_txport]
  Delay10/1(q) -> [gbe_txip]
  Delay72/1(q) -> Subsystem1/1(In1)
  Subsystem1/1(Out1) -> [id0]
  Subsystem1/2(Out2) -> [id1]
  Subsystem1/3(Out3) -> [id2]
  Subsystem1/4(Out4) -> [id3]
  Constant6/1 -> vacc_time_lsw/1(sim_1)
  vacc_time_msw/2(in_msw) -> Concat12/1
  vacc_time_lsw/1(in_reg) -> Concat12/2
  vacc_time_msw/1(in_arm) -> [vacc_ld_arm]
  Concat12/1 -> [vacc_ld_time]
  Delay15/1(q) -> vacc_monitor2/2(eof), [vacc_txeof0], Register/2
  Delay209/1(q) -> negedge_delay5/1(in)
  Delay210/1(q) -> negedge_delay6/1(in)
  negedge_delay6/1(out) -> front_panel/8(led4_green)
  negedge_delay5/1(out) -> front_panel/5(led1_red)
  Delay211/1(q) -> negedge_delay7/1(in)
  negedge_delay7/1(out) -> front_panel/11(led7_green)
  [err0] -> Delay27/1(d)
  [data_in_bad0] -> Inverter3/1
  [data_in_bad1] -> Inverter4/1
  [data_in_bad2] -> Inverter7/1
  [data_in_bad3] -> Inverter8/1
  Inverter3/1 -> Delay210/1(d)
  Inverter4/1 -> Delay118/1(d)
  Inverter7/1 -> Delay17/1(d)
  Inverter8/1 -> Delay211/1(d)
  [err1] -> Delay209/1(d)
  [err2] -> Delay96/1(d)
  [err3] -> Delay97/1(d)
  edge_detect/1(out) -> pipeline1/1(d), pipeline2/1(d)
  pipeline8/1(q) -> [flasher_en]
  pipeline7/1(q) -> [loopback_mux_rst]
  pipeline6/1(q) -> [gbe_out_rst]
  pipeline5/1(q) -> [gbe_out_en]
  pipeline2/1(q) -> [cnt_rst]
  pipeline1/1(q) -> [clr_status]
  pipeline/1(q) -> [vacc_rst]
  tvg_sel/1(in_xaui) -> pipeline9/1(d)
  tvg_sel/2(in_descr) -> pipeline10/1(d)
  tvg_sel/3(in_xeng) -> pipeline12/1(d)
  tvg_sel/4(in_vacc) -> pipeline11/1(d)
  pipeline9/1(q) -> [xaui_tvg_sel]
  pipeline10/1(q) -> [descr_tvg_sel]
  pipeline12/1(q) -> [xeng_tvg_sel]
  pipeline11/1(q) -> [vacc_tvg_sel]
  pipeline13/1(q) -> [gbe_debug_rst]
  gbe0/1(led_up) -> [gbe_up0]
  gbe0/2(led_rx) -> Terminator8/1
  gbe0/3(led_tx) -> Terminator1/1
  gbe0/4(tx_afull) -> Terminator3/1
  gbe0/5(tx_overflow) -> [gbe_tx_over0]
  gbe0/12(rx_overrun) -> Terminator6/1
  gbe0/11(rx_bad_frame) -> [gbe_rx_bad0]
  gbe0/6(rx_data) -> [gbe_rxdata0]
  gbe0/7(rx_valid) -> [gbe_rxvld0]
  gbe0/8(rx_source_ip) -> Terminator4/1
  gbe0/9(rx_source_port) -> Terminator5/1
  gbe0/10(rx_end_of_frame) -> [gbe_rxeof0]
  delay31/1 -> gbe0/1(rst)
  delay32/1 -> gbe0/2(tx_data)
  delay24/1 -> gbe0/3(tx_valid)
  delay25/1 -> gbe0/4(tx_dest_ip)
  delay29/1 -> gbe0/5(tx_dest_port)
  delay30/1 -> gbe0/6(tx_end_of_frame)
  Constant1/1 -> gbe0/7(rx_ack)
  Constant3/1 -> gbe0/8(rx_overrun_ack)
  [gbe_out_rst] -> delay31/1
  [gbe_txd0] -> delay32/1
  [gbe_txvld0] -> delay24/1
  [gbe_txip] -> delay25/1
  [gbe_txport] -> delay29/1
  [gbe_txeof0] -> delay30/1
  [gbe_debug_rst] -> gbe0/9(debug_rst)
  edge_detect1/1(out) -> pipeline7/1(d)
  edge_detect2/1(out) -> pipeline13/1(d)
  [gbe_rxvld0] -> Delay19/1(d)
  [gbe_rxdata0] -> Delay18/1(d)
  [gbe_rxeof0] -> Delay25/1(d)
  Delay18/1(q) -> spead_unpack0/1(pkt_data)
  Delay19/1(q) -> spead_unpack0/2(pkt_valid)
  Delay25/1(q) -> spead_unpack0/3(pkt_eof)
  spead_unpack0/1(pkt_start) -> Terminator7/1
  spead_unpack0/2(data64) -> [spead_data0]
  spead_unpack0/3(valid64) -> [spead_valid0]
  spead_unpack0/4(eof64) -> [spead_eof0]
  spead_unpack0/5(error) -> [spead_error0]
  spead_unpack0/6(hdr_heap_id) -> [spead_heapid0]
  spead_unpack0/7(hdr_heap_size) -> [spead_heapsize0]
  spead_unpack0/8(hdr_heap_offset) -> [spead_heapoffset0]
  spead_unpack0/9(hdr_pkt_len) -> [spead_pktlen0]
  spead_unpack0/10(hdr5_0x1600) -> [spead_hdr1_0]
  spead_unpack0/11(hdr6_0x4101) -> [spead_hdr2_0]
  spead_unpack0/12(hdr7_0x4102) -> [spead_hdr3_0]
  spead_unpack0/13(hdr8_0x4103) -> [spead_hdr4_0]
  Subsystem3/1(rx_cnt) -> Delay29/1(d)
  [cnt_rst] -> Subsystem3/1(rst)
  Subsystem3/2(err_cnt) -> Delay44/1(d)
  Delay29/1(q) -> rx_cnt0/1(out_reg)
  Delay44/1(q) -> rx_err_cnt0/1(out_reg)
  Delay51/1(q) -> Subsystem3/2(we)
  Delay52/1(q) -> Subsystem3/3(eof)
  Delay53/1(q) -> Subsystem3/4(flag)
  [spead_valid0] -> Delay51/1(d)
  [spead_eof0] -> Delay52/1(d)
  [spead_error0] -> Delay53/1(d)
  Slice1/1 -> snap_unpack0/4(in_time)
  Slice2/1 -> snap_unpack0/5(in_feng_id)
  Slice3/1 -> snap_unpack0/6(in_freq)
  Logical2/1 -> snap_unpack0/17(stop)
  [pre_valid_0] -> snap_unpack0/15(we), snap_unpack0/2(in_valid)
  [pre_eof_0] -> snap_unpack0/16(trig), snap_unpack0/3(in_eof)
  [pre_timestamp_0] -> Slice1/1
  [pre_feng_id_0] -> Slice2/1
  [pre_freq_0] -> Slice3/1
  [pre_data_0] -> snap_unpack0/1(in_data)
  [pre_spead_err0] -> Logical2/1
  [pre_rx_dest_err0] -> Logical2/2
  [pre_feng_rx_err0] -> Logical2/3
  [pre_feng_chk_err0] -> Logical2/4
  [pre_feng_rx_err0] -> snap_unpack0/11(in_feng_rx_err)
  [pre_adc_err0] -> snap_unpack0/7(in_adc_over)
  [pre_spead_err0] -> snap_unpack0/8(in_spead_err)
  [pre_rx_dest_err0] -> snap_unpack0/9(in_dest_err)
  [pre_fft_err0] -> snap_unpack0/10(in_fft_err)
  [pre_ndiode_en0] -> snap_unpack0/12(in_nd_en)
  [pre_feng_chk_err0] -> snap_unpack0/13(in_chksum_err)
  [pre_feng_qdr_err0] -> snap_unpack0/14(in_feng_qdr_err)
  pre_process0/9(dest_err) -> [pre_rx_dest_err0]
  pre_process0/8(spead_err_out) -> [pre_spead_err0]
  pre_process0/7(adc_over) -> [pre_adc_err0]
  pre_process0/10(fft_err) -> [pre_fft_err0]
  pre_process0/11(feng_rx_err) -> [pre_feng_rx_err0]
  pre_process0/12(nd_en) -> [pre_ndiode_en0]
  pre_process0/13(chksum_err) -> [pre_feng_chk_err0]
  pre_process0/14(qdr_err) -> [pre_feng_qdr_err0]
  [id0] -> pre_process0/9(board_id)
  [id0] -> pkt_reord_devel0/8(board_id)
  [flags0] -> pkt_reord_devel0/7(flag)
  [spead_data0] -> pre_process0/1(data_in)
  [spead_valid0] -> pre_process0/2(valid_in)
  [spead_eof0] -> pre_process0/3(eof_in)
  [spead_error0] -> pre_process0/4(spead_err)
  [spead_hdr1_0] -> pre_process0/5(hdr1)
  [spead_hdr2_0] -> pre_process0/6(hdr2)
  [spead_hdr3_0] -> pre_process0/7(hdr3)
  [spead_hdr4_0] -> pre_process0/8(hdr4)
  miss_cnt0/2(missing_cnt) -> Convert1/1
  [cnt_rst] -> miss_cnt0/1(rst)
  miss_cnt0/1(spectr_cnt) -> Convert/1
  Delay61/1(q) -> pkt_reord_cnt0/1(out_reg)
  Delay62/1(q) -> pkt_reord_err0/1(out_reg)
  pkt_reord_devel0/4(time_out) -> Slice38/1, Delay26/1(d)
  pkt_reord_devel0/1(sync_out) -> snap_reord0/11(trig), delay61/1, snap_reord0/1(in_sync), Delay20/1(d)
  [xeng_tvg_sel] -> xeng_tvg0/1(tvg_sel)
  Delay20/1(q) -> [xsync_out0], xeng_tvg0/2(sync)
  Delay21/1(q) -> xeng_tvg0/3(data_in)
  Delay130/1(q) -> last_missing_ant0/1(out_reg)
  miss_cnt0/3(last_missed_ant) -> Convert2/1
  pkt_reord_devel0/2(data_out) -> snap_reord0/2(in_data), Delay21/1(d)
  miss_cnt0/4(not_rcvd) -> [xeng_rx_err0]
  pkt_reord_devel0/7(err) -> Terminator9/1
  pkt_reord_devel0/3(valid_out) -> delay62/1, snap_reord0/3(in_valid), snap_reord0/10(we), Logical6/2, Logical28/1, Delay22/1(d)
  pkt_reord_devel0/5(freq_out) -> Convert12/1
  Slice12/1 -> snap_reord0/7(in_feng_err)
  Slice16/1 -> snap_reord0/9(in_nd_on)
  Slice15/1 -> snap_reord0/8(in_adc_over)
  pkt_reord_devel0/6(flag_out) -> Relational16/2, Slice11/1, Slice12/1, Slice15/1, Slice16/1
  Slice11/1 -> Logical6/1, snap_reord0/6(in_xeng_err), delay63/1
  Logical6/1 -> snap_reord0/12(stop)
  Slice38/1 -> snap_reord0/4(in_time)
  Convert12/1 -> snap_reord0/5(in_freq)
  Convert/1 -> Delay61/1(d)
  Convert1/1 -> Delay62/1(d)
  Convert2/1 -> Delay130/1(d)
  Delay22/1(q) -> xeng_tvg0/4(valid_in)
  Delay26/1(q) -> Delay151/1(d)
  delay61/1 -> miss_cnt0/2(sync)
  delay62/1 -> miss_cnt0/3(valid)
  delay63/1 -> miss_cnt0/4(not rcvd)
  xeng_tvg1/1(sync_out) -> Delay32/1(d)
  xeng_tvg1/2(data_out) -> Delay37/1(d)
  xeng_tvg1/3(valid_out) -> Delay38/1(d)
  xeng1/1(sync_out) -> Delay16/1(d)
  xeng1/2(acc) -> Delay49/1(d)
  xeng1/3(valid) -> Delay77/1(d)
  [vacc_tvg_sel] -> vacc_tvg1/1(tvg_sel)
  Delay4/1(q) -> Delay39/1(d)
  16b_32b1/1(Out1) -> snap_xeng1/1(din), vacc_tvg1/3(data_in)
  vacc_tvg1/1(sync_out) -> fake_vacc1/5(sync_in)
  vacc_tvg1/2(data_out) -> fake_vacc1/6(data_in)
  vacc_tvg1/3(valid_out) -> fake_vacc1/7(we)
  [acc_len] -> fake_vacc1/4(acc_len)
  xeng1/4(mcnt_out) -> Delay78/1(d)
  vacc_monitor1/2(spec_cnt) -> vacc_cnt1/1(out_reg)
  vacc_monitor1/1(error_cnt) -> vacc_err_cnt1/1(out_reg)
  fake_vacc1/1(new_acc) -> [new_acc1]
  [cnt_rst] -> vacc_monitor1/1(cnt_rst)
  fake_vacc1/7(timestamp) -> delay13/1
  Delay32/1(q) -> xeng1/1(sync_in)
  Delay37/1(q) -> xeng1/2(ant)
  Delay38/1(q) -> xeng1/3(window_valid)
  Delay39/1(q) -> xeng1/4(mcnt_in)
  [vacc_ld_arm] -> fake_vacc1/2(arm)
  [vacc_ld_time] -> fake_vacc1/3(load_time)
  [vacc_rst] -> fake_vacc1/1(rst)
  delay8/1 -> fake_vacc1/8(pcnt_in)
  fake_vacc1/10(error_out) -> [vacc_err1]
  [new_acc1] -> vacc_monitor1/2(new_acc)
  [vacc_err1] -> vacc_monitor1/3(error)
  fake_vacc1/2(data_out) -> delay3/1
  fake_vacc1/4(valid_out) -> delay1/1
  fake_vacc1/6(rb_done) -> delay9/1
  [vacc_ld_stat1] -> vacc_ld_status1/1(out_reg)
  fake_vacc1/8(ld_status) -> [vacc_ld_stat1]
  [id1] -> pack_out1/6(xeng_id)
  [vacc_err1] -> snap_vacc1/4(stop)
  pack_out1/3(eof) -> Delay3/1(d)
  [cnt_rst] -> vacc_monitor3/1(cnt_rst)
  vacc_monitor3/1(pkt_cnt) -> pack_out_cnt1/1(out_reg)
  vacc_monitor3/2(error_cnt) -> pack_out_err1/1(out_reg)
  pack_out1/5(fetch) -> fake_vacc1/9(re)
  delay3/1 -> snap_vacc1/1(din), pack_out1/1(data_in)
  delay1/1 -> snap_vacc1/2(we), pack_out1/2(valid_in)
  delay9/1 -> snap_vacc1/3(trig), pack_out1/4(rb_done)
  delay13/1 -> pack_out1/5(timestamp)
  pack_out1/1(data_out) -> Delay14/1(d)
  pack_out1/4(err) -> Delay28/1(d)
  Delay28/1(q) -> vacc_monitor3/3(error), [pack_err1]
  Logical1/1 -> [vacc_txvld1]
  Delay14/1(q) -> [vacc_txd1]
  pre_process0/1(data_out) -> [pre_data_0], pkt_reord_devel0/1(din)
  pre_process0/2(valid) -> [pre_valid_0], pkt_reord_devel0/2(valid_in)
  pre_process0/3(eof_out) -> [pre_eof_0], pkt_reord_devel0/3(eof)
  pre_process0/4(timestamp) -> pkt_reord_devel0/4(time), [pre_timestamp_0]
  pre_process0/5(feng_id) -> pkt_reord_devel0/5(ant), [pre_feng_id_0]
  pre_process0/6(freq_out) -> pkt_reord_devel0/6(freq), [pre_freq_0]
  [id1] -> pkt_reord_devel1/8(board_id)
  [flags1] -> pkt_reord_devel1/7(flag)
  miss_cnt1/2(missing_cnt) -> Convert4/1
  [cnt_rst] -> miss_cnt1/1(rst)
  miss_cnt1/1(spectr_cnt) -> Convert3/1
  Delay33/1(q) -> pkt_reord_cnt1/1(out_reg)
  Delay36/1(q) -> pkt_reord_err1/1(out_reg)
  pkt_reord_devel1/4(time_out) -> Slice8/1, Delay24/1(d)
  pkt_reord_devel1/1(sync_out) -> snap_reord1/11(trig), delay10/1, snap_reord1/1(in_sync), Delay6/1(d)
  [xeng_tvg_sel] -> xeng_tvg1/1(tvg_sel)
  Delay6/1(q) -> xeng_tvg1/2(sync)
  Delay7/1(q) -> xeng_tvg1/3(data_in)
  Delay2/1(q) -> last_missing_ant1/1(out_reg)
  miss_cnt1/3(last_missed_ant) -> Convert13/1
  pkt_reord_devel1/2(data_out) -> snap_reord1/2(in_data), Delay7/1(d)
  miss_cnt1/4(not_rcvd) -> [xeng_rx_err1]
  pkt_reord_devel1/7(err) -> Terminator2/1
  pkt_reord_devel1/5(freq_out) -> Convert5/1
  Slice5/1 -> snap_reord1/7(in_feng_err)
  Slice7/1 -> snap_reord1/9(in_nd_on)
  Slice6/1 -> snap_reord1/8(in_adc_over)
  Slice4/1 -> Logical3/1, snap_reord1/6(in_xeng_err), delay12/1
  Logical3/1 -> snap_reord1/12(stop)
  Slice8/1 -> snap_reord1/4(in_time)
  Convert5/1 -> snap_reord1/5(in_freq)
  Convert3/1 -> Delay33/1(d)
  Convert4/1 -> Delay36/1(d)
  Convert13/1 -> Delay2/1(d)
  Delay11/1(q) -> xeng_tvg1/4(valid_in)
  Delay24/1(q) -> Delay4/1(d)
  delay10/1 -> miss_cnt1/2(sync)
  delay11/1 -> miss_cnt1/3(valid)
  delay12/1 -> miss_cnt1/4(not rcvd)
  Slice9/1 -> snap_unpack1/4(in_time)
  Slice10/1 -> snap_unpack1/5(in_feng_id)
  Slice13/1 -> snap_unpack1/6(in_freq)
  Logical4/1 -> snap_unpack1/17(stop)
  [pre_valid_1] -> snap_unpack1/15(we), snap_unpack1/2(in_valid)
  [pre_eof_1] -> snap_unpack1/16(trig), snap_unpack1/3(in_eof)
  [pre_timestamp_1] -> Slice9/1
  [pre_feng_id_1] -> Slice10/1
  [pre_freq_1] -> Slice13/1
  [pre_data_1] -> snap_unpack1/1(in_data)
  [pre_spead_err1] -> Logical4/1
  [pre_rx_dest_err1] -> Logical4/2
  [pre_feng_rx_err1] -> Logical4/3
  [pre_feng_chk_err1] -> Logical4/4
  [pre_feng_rx_err1] -> snap_unpack1/11(in_feng_rx_err)
  [pre_adc_err1] -> snap_unpack1/7(in_adc_over)
  [pre_spead_err1] -> snap_unpack1/8(in_spead_err)
  [pre_rx_dest_err1] -> snap_unpack1/9(in_dest_err)
  [pre_fft_err1] -> snap_unpack1/10(in_fft_err)
  [pre_ndiode_en1] -> snap_unpack1/12(in_nd_en)
  [pre_feng_chk_err1] -> snap_unpack1/13(in_chksum_err)
  [pre_feng_qdr_err1] -> snap_unpack1/14(in_feng_qdr_err)
  pre_process1/9(dest_err) -> [pre_rx_dest_err1]
  pre_process1/8(spead_err_out) -> [pre_spead_err1]
  pre_process1/7(adc_over) -> [pre_adc_err1]
  pre_process1/10(fft_err) -> [pre_fft_err1]
  pre_process1/11(feng_rx_err) -> [pre_feng_rx_err1]
  pre_process1/12(nd_en) -> [pre_ndiode_en1]
  pre_process1/13(chksum_err) -> [pre_feng_chk_err1]
  pre_process1/14(qdr_err) -> [pre_feng_qdr_err1]
  [id1] -> pre_process1/9(board_id)
  [spead_data0] -> pre_process1/1(data_in)
  [spead_valid0] -> pre_process1/2(valid_in)
  [spead_eof0] -> pre_process1/3(eof_in)
  [spead_error0] -> pre_process1/4(spead_err)
  [spead_hdr1_0] -> pre_process1/5(hdr1)
  [spead_hdr2_0] -> pre_process1/6(hdr2)
  [spead_hdr3_0] -> pre_process1/7(hdr3)
  [spead_hdr4_0] -> pre_process1/8(hdr4)
  pre_process1/1(data_out) -> pkt_reord_devel1/1(din), [pre_data_1]
  pre_process1/2(valid) -> pkt_reord_devel1/2(valid_in), [pre_valid_1]
  pre_process1/3(eof_out) -> pkt_reord_devel1/3(eof), [pre_eof_1]
  pre_process1/4(timestamp) -> pkt_reord_devel1/4(time), [pre_timestamp_1]
  pre_process1/5(feng_id) -> pkt_reord_devel1/5(ant), [pre_feng_id_1]
  pre_process1/6(freq_out) -> pkt_reord_devel1/6(freq), [pre_freq_1]
  [pre_freq_0] -> Slice/1
  Constant/1 -> Relational/2
  [pre_feng_id_0] -> Slice20/1
  Relational/1 -> Logical5/2
  Logical5/1 -> delay47/1
  Convert18/1 -> Delay40/1(d)
  highwater16/1(highmark) -> Convert18/1
  Delay40/1(q) -> highmark0_01/1(out_high0)
  Convert19/1 -> Delay41/1(d)
  Delay41/1(q) -> highmark0_01/2(out_high1)
  Convert16/1 -> Delay42/1(d)
  Convert17/1 -> Delay54/1(d)
  Delay42/1(q) -> highmark0_23/1(out_high2)
  Delay54/1(q) -> highmark0_23/2(out_high3)
  delay16/1 -> highwater16/1(reset)
  delay46/1 -> highwater16/3(data)
  delay47/1 -> highwater16/2(valid)
  Constant2/1 -> Relational1/2
  Relational1/1 -> Logical7/2
  Logical7/1 -> delay35/1
  delay17/1 -> highwater1/1(reset)
  delay18/1 -> highwater1/3(data)
  delay35/1 -> highwater1/2(valid)
  highwater1/1(highmark) -> Convert19/1
  Constant4/1 -> Relational2/2
  Relational2/1 -> Logical8/2
  Logical8/1 -> delay43/1
  delay42/1 -> highwater3/3(data)
  delay43/1 -> highwater3/2(valid)
  Slice/1 -> delay18/1, delay40/1, delay42/1, delay46/1
  Constant5/1 -> Relational3/2
  Relational3/1 -> Logical9/2
  Logical9/1 -> delay41/1
  [pre_valid_0] -> Logical8/1, Logical9/1, Logical7/1, Logical5/1
  delay36/1 -> highwater2/1(reset)
  delay40/1 -> highwater2/3(data)
  delay41/1 -> highwater2/2(valid)
  [cnt_rst] -> delay17/1, delay45/1, delay36/1, delay16/1
  Slice20/1 -> Relational2/1, Relational3/1, Relational1/1, Relational/1
  [id0] -> highwater3/4(xid), highwater2/4(xid), highwater1/4(xid), highwater16/4(xid)
  delay45/1 -> highwater3/1(reset)
  highwater3/1(highmark) -> Convert16/1
  highwater2/1(highmark) -> Convert17/1
  [pre_freq_1] -> Slice14/1
  Constant7/1 -> Relational4/2
  [pre_feng_id_1] -> Slice17/1
  Relational4/1 -> Logical10/2
  Logical10/1 -> delay59/1
  Convert22/1 -> Delay55/1(d)
  highwater5/1(highmark) -> Convert22/1
  Delay55/1(q) -> highmark1_01/1(out_high0)
  Convert23/1 -> Delay57/1(d)
  Delay57/1(q) -> highmark1_01/2(out_high1)
  Convert20/1 -> Delay58/1(d)
  Convert21/1 -> Delay59/1(d)
  Delay58/1(q) -> highmark1_23/1(out_high2)
  Delay59/1(q) -> highmark1_23/2(out_high3)
  delay48/1 -> highwater5/1(reset)
  delay58/1 -> highwater5/3(data)
  delay59/1 -> highwater5/2(valid)
  Constant8/1 -> Relational5/2
  Relational5/1 -> Logical11/2
  Logical11/1 -> delay51/1
  delay49/1 -> highwater4/1(reset)
  delay50/1 -> highwater4/3(data)
  delay51/1 -> highwater4/2(valid)
  highwater4/1(highmark) -> Convert23/1
  Constant10/1 -> Relational6/2
  Relational6/1 -> Logical14/2
  Logical14/1 -> delay56/1
  delay55/1 -> highwater7/3(data)
  delay56/1 -> highwater7/2(valid)
  Slice14/1 -> delay58/1, delay55/1, delay53/1, delay50/1
  Constant11/1 -> Relational7/2
  Relational7/1 -> Logical15/2
  Logical15/1 -> delay54/1
  [pre_valid_1] -> Logical10/1, Logical11/1, Logical15/1, Logical14/1
  delay52/1 -> highwater6/1(reset)
  delay53/1 -> highwater6/3(data)
  delay54/1 -> highwater6/2(valid)
  [cnt_rst] -> delay48/1, delay49/1, delay52/1, delay57/1
  Slice17/1 -> Relational4/1, Relational5/1, Relational7/1, Relational6/1
  [id1] -> highwater5/4(xid), highwater4/4(xid), highwater6/4(xid), highwater7/4(xid)
  delay57/1 -> highwater7/1(reset)
  highwater7/1(highmark) -> Convert20/1
  highwater6/1(highmark) -> Convert21/1
  Concat/1 -> gbe_mux_bus0/1(di)
  [vacc_txd1] -> Concat/2
  [vacc_txd0] -> Concat/1
  [vacc_txvld1] -> Concat1/2
  [vacc_txvld0] -> Concat1/1
  Concat1/1 -> gbe_mux_bus0/2(validi)
  [vacc_txeof1] -> Concat2/2
  [vacc_txeof0] -> Concat2/1
  Concat2/1 -> gbe_mux_bus0/3(eofi)
  fake_vacc0/5(pkt_rdy) -> [vacc_ready0]
  fake_vacc1/5(pkt_rdy) -> [vacc_ready1]
  gbe_mux_bus0/5(start) -> bus_expand/1(bus_in)
  bus_expand/1(msb_out2) -> [go0]
  bus_expand/2(lsb_out1) -> [go1]
  Concat3/1 -> gbe_mux_bus0/4(drdy)
  [vacc_ready0] -> Concat3/1
  [vacc_ready1] -> Concat3/2
  gbe_mux_bus0/2(do) -> [gbe_txd0]
  gbe_mux_bus0/3(valido) -> [gbe_txvld0]
  gbe_mux_bus0/4(eofo) -> [gbe_txeof0]
  gbe_mux_bus0/1(input) -> Terminator/1
  xeng_tvg2/1(sync_out) -> Delay102/1(d)
  xeng_tvg2/2(data_out) -> Delay110/1(d)
  xeng_tvg2/3(valid_out) -> Delay111/1(d)
  xeng2/1(sync_out) -> Delay92/1(d)
  xeng2/2(acc) -> Delay93/1(d)
  xeng2/3(valid) -> Delay94/1(d)
  [vacc_tvg_sel] -> vacc_tvg2/1(tvg_sel)
  Delay48/1(q) -> Delay112/1(d)
  16b_32b2/1(Out1) -> vacc_tvg2/3(data_in), snap_xeng2/1(din)
  vacc_tvg2/1(sync_out) -> fake_vacc2/5(sync_in)
  vacc_tvg2/2(data_out) -> fake_vacc2/6(data_in)
  vacc_tvg2/3(valid_out) -> fake_vacc2/7(we)
  [acc_len] -> fake_vacc2/4(acc_len)
  xeng2/4(mcnt_out) -> Delay113/1(d)
  vacc_monitor4/2(spec_cnt) -> vacc_cnt2/1(out_reg)
  vacc_monitor4/1(error_cnt) -> vacc_err_cnt2/1(out_reg)
  fake_vacc2/1(new_acc) -> [new_acc2]
  [cnt_rst] -> vacc_monitor4/1(cnt_rst)
  fake_vacc2/7(timestamp) -> delay90/1
  Delay102/1(q) -> xeng2/1(sync_in)
  Delay110/1(q) -> xeng2/2(ant)
  Delay111/1(q) -> xeng2/3(window_valid)
  Delay112/1(q) -> xeng2/4(mcnt_in)
  [vacc_ld_arm] -> fake_vacc2/2(arm)
  [vacc_ld_time] -> fake_vacc2/3(load_time)
  [vacc_rst] -> fake_vacc2/1(rst)
  delay75/1 -> fake_vacc2/8(pcnt_in)
  fake_vacc2/10(error_out) -> [vacc_err2]
  [new_acc2] -> vacc_monitor4/2(new_acc)
  [vacc_err2] -> vacc_monitor4/3(error)
  fake_vacc2/2(data_out) -> delay65/1
  fake_vacc2/4(valid_out) -> delay27/1
  fake_vacc2/6(rb_done) -> delay86/1
  [vacc_ld_stat2] -> vacc_ld_status2/1(out_reg)
  fake_vacc2/8(ld_status) -> [vacc_ld_stat2]
  [id2] -> pack_out2/6(xeng_id)
  [vacc_err2] -> snap_vacc2/4(stop)
  pack_out2/3(eof) -> Delay47/1(d)
  [cnt_rst] -> vacc_monitor6/1(cnt_rst)
  vacc_monitor6/1(pkt_cnt) -> pack_out_cnt2/1(out_reg)
  vacc_monitor6/2(error_cnt) -> pack_out_err2/1(out_reg)
  pack_out2/5(fetch) -> fake_vacc2/9(re)
  delay65/1 -> pack_out2/1(data_in), snap_vacc2/1(din)
  delay27/1 -> pack_out2/2(valid_in), snap_vacc2/2(we)
  delay86/1 -> pack_out2/4(rb_done), snap_vacc2/3(trig)
  delay90/1 -> pack_out2/5(timestamp)
  pack_out2/1(data_out) -> Delay67/1(d)
  pack_out2/4(err) -> Delay81/1(d)
  Delay81/1(q) -> [pack_err2], vacc_monitor6/3(error)
  [gbe_up1] -> Inverter2/1
  latch2/17(data_bad) -> [data_in_bad2]
  latch2/18(error) -> [err2]
  latch2/19(flags) -> [flags2]
  [gbe_up1] -> Inverter1/1
  [clr_status] -> latch3/1(reset)
  [pack_err3] -> latch3/15(pack_err)
  latch3/12(Out12) -> status3/12(out_tx_over)
  latch3/14(Out14) -> status3/14(out_pack_err)
  latch3/10(Out10) -> status3/10(out_rx_bad_pkt)
  latch3/11(Out11) -> status3/11(out_rx_bad_frame)
  latch3/9(Out9) -> status3/9(out_vacc_err)
  latch3/13(Out13) -> status3/13(out_xeng_bad_dat)
  latch3/4(Out4) -> status3/4(out_fft_err)
  latch3/6(Out6) -> status3/6(out_feng_chk_err)
  latch3/8(Out8) -> status3/8(out_noise_diode_en)
  latch3/7(Out7) -> status3/7(out_adc_over)
  latch3/3(Out3) -> status3/3(out_feng_rx_err)
  latch3/2(Out2) -> status3/2(out_rx_dest_err)
  latch3/5(Out5) -> status3/5(out_feng_qdr_err)
  latch3/1(Out1) -> status3/1(out_gbe_down)
  latch3/17(data_bad) -> [data_in_bad3]
  latch3/18(error) -> [err3]
  latch3/19(flags) -> [flags3]
  Inverter1/1 -> latch3/2(gbe_down)
  [pre_rx_dest_err3] -> latch3/3(rx_dest_err)
  [pre_feng_rx_err3] -> latch3/4(feng_rx_err)
  [pre_ndiode_en3] -> latch3/9(noise_diode_en)
  [pre_adc_err3] -> latch3/8(adc_over)
  [vacc_err3] -> latch3/10(vacc_err)
  [pre_spead_err3] -> latch3/11(rx_bad_pkt)
  [pre_feng_chk_err3] -> latch3/7(feng_chk_err)
  [gbe_rx_bad1] -> latch3/12(rx_bad_frame)
  [pre_feng_qdr_err3] -> latch3/6(feng_qdr_err)
  [gbe_tx_over1] -> latch3/13(tx_over)
  [pre_fft_err3] -> latch3/5(fft_err)
  [xeng_rx_err3] -> latch3/14(xeng_bad_dat)
  gbe1/1(led_up) -> [gbe_up1]
  gbe1/2(led_rx) -> Terminator18/1
  gbe1/3(led_tx) -> Terminator11/1
  gbe1/4(tx_afull) -> Terminator13/1
  gbe1/5(tx_overflow) -> [gbe_tx_over1]
  gbe1/12(rx_overrun) -> Terminator16/1
  gbe1/11(rx_bad_frame) -> [gbe_rx_bad1]
  gbe1/6(rx_data) -> [gbe_rxdata1]
  gbe1/7(rx_valid) -> [gbe_rxvld1]
  gbe1/8(rx_source_ip) -> Terminator14/1
  gbe1/9(rx_source_port) -> Terminator15/1
  gbe1/10(rx_end_of_frame) -> [gbe_rxeof1]
  delay39/1 -> gbe1/1(rst)
  delay44/1 -> gbe1/2(tx_data)
  delay28/1 -> gbe1/3(tx_valid)
  delay33/1 -> gbe1/4(tx_dest_ip)
  delay34/1 -> gbe1/5(tx_dest_port)
  delay38/1 -> gbe1/6(tx_end_of_frame)
  Constant12/1 -> gbe1/7(rx_ack)
  Constant16/1 -> gbe1/8(rx_overrun_ack)
  [gbe_out_rst] -> delay39/1
  [gbe_txd1] -> delay44/1
  [gbe_txvld1] -> delay28/1
  [gbe_txip] -> delay33/1
  [gbe_txport] -> delay34/1
  [gbe_txeof1] -> delay38/1
  [gbe_debug_rst] -> gbe1/9(debug_rst)
  [gbe_rxvld1] -> Delay60/1(d)
  [gbe_rxdata1] -> Delay50/1(d)
  [gbe_rxeof1] -> Delay69/1(d)
  Delay50/1(q) -> spead_unpack1/1(pkt_data)
  Delay60/1(q) -> spead_unpack1/2(pkt_valid)
  Delay69/1(q) -> spead_unpack1/3(pkt_eof)
  spead_unpack1/1(pkt_start) -> Terminator17/1
  spead_unpack1/2(data64) -> [spead_data1]
  spead_unpack1/3(valid64) -> [spead_valid1]
  spead_unpack1/4(eof64) -> [spead_eof1]
  spead_unpack1/5(error) -> [spead_error1]
  spead_unpack1/6(hdr_heap_id) -> [spead_heapid1]
  spead_unpack1/7(hdr_heap_size) -> [spead_heapsize1]
  spead_unpack1/8(hdr_heap_offset) -> [spead_heapoffset1]
  spead_unpack1/9(hdr_pkt_len) -> [spead_pktlen1]
  spead_unpack1/10(hdr5_0x1600) -> [spead_hdr1_1]
  spead_unpack1/11(hdr6_0x4101) -> [spead_hdr2_1]
  spead_unpack1/12(hdr7_0x4102) -> [spead_hdr3_1]
  spead_unpack1/13(hdr8_0x4103) -> [spead_hdr4_1]
  Subsystem4/1(rx_cnt) -> Delay75/1(d)
  [cnt_rst] -> Subsystem4/1(rst)
  Subsystem4/2(err_cnt) -> Delay91/1(d)
  Delay75/1(q) -> rx_cnt1/1(out_reg)
  Delay91/1(q) -> rx_err_cnt1/1(out_reg)
  Delay95/1(q) -> Subsystem4/2(we)
  Delay98/1(q) -> Subsystem4/3(eof)
  Delay99/1(q) -> Subsystem4/4(flag)
  [spead_valid1] -> Delay95/1(d)
  [spead_eof1] -> Delay98/1(d)
  [spead_error1] -> Delay99/1(d)
  Slice19/1 -> snap_unpack2/4(in_time)
  Slice29/1 -> snap_unpack2/5(in_feng_id)
  Slice31/1 -> snap_unpack2/6(in_freq)
  Logical20/1 -> snap_unpack2/17(stop)
  [pre_valid_2] -> snap_unpack2/2(in_valid), snap_unpack2/15(we)
  [pre_eof_2] -> snap_unpack2/3(in_eof), snap_unpack2/16(trig)
  [pre_timestamp_2] -> Slice19/1
  [pre_feng_id_2] -> Slice29/1
  [pre_freq_2] -> Slice31/1
  [pre_data_2] -> snap_unpack2/1(in_data)
  [pre_spead_err2] -> Logical20/1
  [pre_rx_dest_err2] -> Logical20/2
  [pre_feng_rx_err2] -> Logical20/3
  [pre_feng_chk_err2] -> Logical20/4
  [pre_feng_rx_err2] -> snap_unpack2/11(in_feng_rx_err)
  [pre_adc_err2] -> snap_unpack2/7(in_adc_over)
  [pre_spead_err2] -> snap_unpack2/8(in_spead_err)
  [pre_rx_dest_err2] -> snap_unpack2/9(in_dest_err)
  [pre_fft_err2] -> snap_unpack2/10(in_fft_err)
  [pre_ndiode_en2] -> snap_unpack2/12(in_nd_en)
  [pre_feng_chk_err2] -> snap_unpack2/13(in_chksum_err)
  [pre_feng_qdr_err2] -> snap_unpack2/14(in_feng_qdr_err)
  pre_process2/9(dest_err) -> [pre_rx_dest_err2]
  pre_process2/8(spead_err_out) -> [pre_spead_err2]
  pre_process2/7(adc_over) -> [pre_adc_err2]
  pre_process2/10(fft_err) -> [pre_fft_err2]
  pre_process2/11(feng_rx_err) -> [pre_feng_rx_err2]
  pre_process2/12(nd_en) -> [pre_ndiode_en2]
  pre_process2/13(chksum_err) -> [pre_feng_chk_err2]
  pre_process2/14(qdr_err) -> [pre_feng_qdr_err2]
  [id2] -> pre_process2/9(board_id)
  [id2] -> pkt_reord_devel2/8(board_id)
  [flags2] -> pkt_reord_devel2/7(flag)
  [spead_data1] -> pre_process2/1(data_in)
  [spead_valid1] -> pre_process2/2(valid_in)
  [spead_eof1] -> pre_process2/3(eof_in)
  [spead_error1] -> pre_process2/4(spead_err)
  [spead_hdr1_1] -> pre_process2/5(hdr1)
  [spead_hdr2_1] -> pre_process2/6(hdr2)
  [spead_hdr3_1] -> pre_process2/7(hdr3)
  [spead_hdr4_1] -> pre_process2/8(hdr4)
  miss_cnt2/2(missing_cnt) -> Convert7/1
  [cnt_rst] -> miss_cnt2/1(rst)
  miss_cnt2/1(spectr_cnt) -> Convert6/1
  Delay107/1(q) -> pkt_reord_cnt2/1(out_reg)
  Delay108/1(q) -> pkt_reord_err2/1(out_reg)
  pkt_reord_devel2/4(time_out) -> Delay70/1(d), Slice32/1
  pkt_reord_devel2/1(sync_out) -> Delay64/1(d), snap_reord2/1(in_sync), delay87/1, snap_reord2/11(trig)
  [xeng_tvg_sel] -> xeng_tvg2/1(tvg_sel)
  Delay64/1(q) -> xeng_tvg2/2(sync)
  Delay65/1(q) -> xeng_tvg2/3(data_in)
  Delay35/1(q) -> last_missing_ant2/1(out_reg)
  miss_cnt2/3(last_missed_ant) -> Convert24/1
  pkt_reord_devel2/2(data_out) -> Delay65/1(d), snap_reord2/2(in_data)
  miss_cnt2/4(not_rcvd) -> [xeng_rx_err2]
  pkt_reord_devel2/7(err) -> Terminator19/1
  pkt_reord_devel2/3(valid_out) -> Logical30/1, Delay66/1(d), Logical24/2, snap_reord2/10(we), snap_reord2/3(in_valid), delay88/1
  pkt_reord_devel2/5(freq_out) -> Convert8/1
  Slice23/1 -> snap_reord2/7(in_feng_err)
  Slice27/1 -> snap_reord2/9(in_nd_on)
  Slice26/1 -> snap_reord2/8(in_adc_over)
  Slice22/1 -> delay89/1, snap_reord2/6(in_xeng_err), Logical24/1
  Logical24/1 -> snap_reord2/12(stop)
  Slice32/1 -> snap_reord2/4(in_time)
  Convert8/1 -> snap_reord2/5(in_freq)
  Convert6/1 -> Delay107/1(d)
  Convert7/1 -> Delay108/1(d)
  Convert24/1 -> Delay35/1(d)
  Delay66/1(q) -> xeng_tvg2/4(valid_in)
  Delay70/1(q) -> Delay48/1(d)
  delay87/1 -> miss_cnt2/2(sync)
  delay88/1 -> miss_cnt2/3(valid)
  delay89/1 -> miss_cnt2/4(not rcvd)
  xeng_tvg3/1(sync_out) -> Delay79/1(d)
  xeng_tvg3/2(data_out) -> Delay84/1(d)
  xeng_tvg3/3(valid_out) -> Delay85/1(d)
  xeng3/1(sync_out) -> Delay114/1(d)
  xeng3/2(acc) -> Delay115/1(d)
  xeng3/3(valid) -> Delay116/1(d)
  [vacc_tvg_sel] -> vacc_tvg3/1(tvg_sel)
  Delay87/1(q) -> Delay86/1(d)
  16b_32b3/1(Out1) -> vacc_tvg3/3(data_in), snap_xeng3/1(din)
  vacc_tvg3/1(sync_out) -> fake_vacc3/5(sync_in)
  vacc_tvg3/2(data_out) -> fake_vacc3/6(data_in)
  vacc_tvg3/3(valid_out) -> fake_vacc3/7(we)
  [acc_len] -> fake_vacc3/4(acc_len)
  xeng3/4(mcnt_out) -> Delay117/1(d)
  vacc_monitor5/2(spec_cnt) -> vacc_cnt3/1(out_reg)
  vacc_monitor5/1(error_cnt) -> vacc_err_cnt3/1(out_reg)
  fake_vacc3/1(new_acc) -> [new_acc3]
  [cnt_rst] -> vacc_monitor5/1(cnt_rst)
  fake_vacc3/7(timestamp) -> delay21/1
  Delay79/1(q) -> xeng3/1(sync_in)
  Delay84/1(q) -> xeng3/2(ant)
  Delay85/1(q) -> xeng3/3(window_valid)
  Delay86/1(q) -> xeng3/4(mcnt_in)
  [vacc_ld_arm] -> fake_vacc3/2(arm)
  [vacc_ld_time] -> fake_vacc3/3(load_time)
  [vacc_rst] -> fake_vacc3/1(rst)
  delay91/1 -> fake_vacc3/8(pcnt_in)
  fake_vacc3/10(error_out) -> [vacc_err3]
  [new_acc3] -> vacc_monitor5/2(new_acc)
  [vacc_err3] -> vacc_monitor5/3(error)
  fake_vacc3/2(data_out) -> delay37/1
  fake_vacc3/4(valid_out) -> delay14/1
  fake_vacc3/6(rb_done) -> delay92/1
  [vacc_ld_stat3] -> vacc_ld_status3/1(out_reg)
  fake_vacc3/8(ld_status) -> [vacc_ld_stat3]
  [id3] -> pack_out3/6(xeng_id)
  [vacc_err3] -> snap_vacc3/4(stop)
  pack_out3/3(eof) -> Delay76/1(d)
  [cnt_rst] -> vacc_monitor7/1(cnt_rst)
  vacc_monitor7/1(pkt_cnt) -> pack_out_cnt3/1(out_reg)
  vacc_monitor7/2(error_cnt) -> pack_out_err3/1(out_reg)
  pack_out3/5(fetch) -> fake_vacc3/9(re)
  delay37/1 -> pack_out3/1(data_in), snap_vacc3/1(din)
  delay14/1 -> pack_out3/2(valid_in), snap_vacc3/2(we)
  delay92/1 -> pack_out3/4(rb_done), snap_vacc3/3(trig)
  delay21/1 -> pack_out3/5(timestamp)
  pack_out3/1(data_out) -> Delay43/1(d)
  pack_out3/4(err) -> Delay71/1(d)
  Delay71/1(q) -> [pack_err3], vacc_monitor7/3(error)
  Logical13/1 -> [vacc_txvld3]
  Delay43/1(q) -> [vacc_txd3]
  pre_process2/1(data_out) -> pkt_reord_devel2/1(din), [pre_data_2]
  pre_process2/2(valid) -> pkt_reord_devel2/2(valid_in), [pre_valid_2]
  pre_process2/3(eof_out) -> pkt_reord_devel2/3(eof), [pre_eof_2]
  pre_process2/4(timestamp) -> [pre_timestamp_2], pkt_reord_devel2/4(time)
  pre_process2/5(feng_id) -> [pre_feng_id_2], pkt_reord_devel2/5(ant)
  pre_process2/6(freq_out) -> [pre_freq_2], pkt_reord_devel2/6(freq)
  [id3] -> pkt_reord_devel3/8(board_id)
  [flags3] -> pkt_reord_devel3/7(flag)
  miss_cnt3/2(missing_cnt) -> Convert30/1
  [cnt_rst] -> miss_cnt3/1(rst)
  miss_cnt3/1(spectr_cnt) -> Convert29/1
  Delay80/1(q) -> pkt_reord_cnt3/1(out_reg)
  Delay82/1(q) -> pkt_reord_err3/1(out_reg)
  pkt_reord_devel3/4(time_out) -> Delay68/1(d), Slice37/1
  pkt_reord_devel3/1(sync_out) -> Delay106/1(d), snap_reord3/1(in_sync), delay15/1, snap_reord3/11(trig)
  [xeng_tvg_sel] -> xeng_tvg3/1(tvg_sel)
  Delay106/1(q) -> xeng_tvg3/2(sync)
  Delay109/1(q) -> xeng_tvg3/3(data_in)
  Delay63/1(q) -> last_missing_ant3/1(out_reg)
  miss_cnt3/3(last_missed_ant) -> Convert9/1
  pkt_reord_devel3/2(data_out) -> Delay109/1(d), snap_reord3/2(in_data)
  miss_cnt3/4(not_rcvd) -> [xeng_rx_err3]
  pkt_reord_devel3/7(err) -> Terminator12/1
  pkt_reord_devel3/3(valid_out) -> Delay12/1(d), Logical31/1, Logical21/2, snap_reord3/10(we), snap_reord3/3(in_valid), delay19/1
  pkt_reord_devel3/5(freq_out) -> Convert31/1
  Slice34/1 -> snap_reord3/7(in_feng_err)
  Slice36/1 -> snap_reord3/9(in_nd_on)
  Slice35/1 -> snap_reord3/8(in_adc_over)
  Slice33/1 -> delay20/1, snap_reord3/6(in_xeng_err), Logical21/1
  Logical21/1 -> snap_reord3/12(stop)
  Slice37/1 -> snap_reord3/4(in_time)
  Convert31/1 -> snap_reord3/5(in_freq)
  Convert29/1 -> Delay80/1(d)
  Convert30/1 -> Delay82/1(d)
  Convert9/1 -> Delay63/1(d)
  Delay12/1(q) -> xeng_tvg3/4(valid_in)
  Delay68/1(q) -> Delay87/1(d)
  delay15/1 -> miss_cnt3/2(sync)
  delay19/1 -> miss_cnt3/3(valid)
  delay20/1 -> miss_cnt3/4(not rcvd)
  Slice39/1 -> snap_unpack3/4(in_time)
  Slice21/1 -> snap_unpack3/5(in_feng_id)
  Slice24/1 -> snap_unpack3/6(in_freq)
  Logical22/1 -> snap_unpack3/17(stop)
  [pre_valid_3] -> snap_unpack3/2(in_valid), snap_unpack3/15(we)
  [pre_eof_3] -> snap_unpack3/3(in_eof), snap_unpack3/16(trig)
  [pre_timestamp_3] -> Slice39/1
  [pre_feng_id_3] -> Slice21/1
  [pre_freq_3] -> Slice24/1
  [pre_data_3] -> snap_unpack3/1(in_data)
  [pre_spead_err3] -> Logical22/1
  [pre_rx_dest_err3] -> Logical22/2
  [pre_feng_rx_err3] -> Logical22/3
  [pre_feng_chk_err3] -> Logical22/4
  [pre_feng_rx_err3] -> snap_unpack3/11(in_feng_rx_err)
  [pre_adc_err3] -> snap_unpack3/7(in_adc_over)
  [pre_spead_err3] -> snap_unpack3/8(in_spead_err)
  [pre_rx_dest_err3] -> snap_unpack3/9(in_dest_err)
  [pre_fft_err3] -> snap_unpack3/10(in_fft_err)
  [pre_ndiode_en3] -> snap_unpack3/12(in_nd_en)
  [pre_feng_chk_err3] -> snap_unpack3/13(in_chksum_err)
  [pre_feng_qdr_err3] -> snap_unpack3/14(in_feng_qdr_err)
  pre_process3/9(dest_err) -> [pre_rx_dest_err3]
  pre_process3/8(spead_err_out) -> [pre_spead_err3]
  pre_process3/7(adc_over) -> [pre_adc_err3]
  pre_process3/10(fft_err) -> [pre_fft_err3]
  pre_process3/11(feng_rx_err) -> [pre_feng_rx_err3]
  pre_process3/12(nd_en) -> [pre_ndiode_en3]
  pre_process3/13(chksum_err) -> [pre_feng_chk_err3]
  pre_process3/14(qdr_err) -> [pre_feng_qdr_err3]
  [spead_data1] -> pre_process3/1(data_in)
  [spead_valid1] -> pre_process3/2(valid_in)
  [spead_eof1] -> pre_process3/3(eof_in)
  [spead_error1] -> pre_process3/4(spead_err)
  [spead_hdr1_1] -> pre_process3/5(hdr1)
  [spead_hdr2_1] -> pre_process3/6(hdr2)
  [spead_hdr3_1] -> pre_process3/7(hdr3)
  [spead_hdr4_1] -> pre_process3/8(hdr4)
  pre_process3/1(data_out) -> [pre_data_3], pkt_reord_devel3/1(din)
  pre_process3/2(valid) -> [pre_valid_3], pkt_reord_devel3/2(valid_in)
  pre_process3/3(eof_out) -> [pre_eof_3], pkt_reord_devel3/3(eof)
  pre_process3/4(timestamp) -> [pre_timestamp_3], pkt_reord_devel3/4(time)
  pre_process3/5(feng_id) -> [pre_feng_id_3], pkt_reord_devel3/5(ant)
  pre_process3/6(freq_out) -> [pre_freq_3], pkt_reord_devel3/6(freq)
  [pre_freq_2] -> Slice18/1
  Constant9/1 -> Relational8/2
  [pre_feng_id_2] -> Slice30/1
  Relational8/1 -> Logical23/2
  Logical23/1 -> delay72/1
  Convert14/1 -> Delay88/1(d)
  highwater9/1(highmark) -> Convert14/1
  Delay88/1(q) -> highmark2_01/1(out_high0)
  Convert15/1 -> Delay89/1(d)
  Delay89/1(q) -> highmark2_01/2(out_high1)
  Convert10/1 -> Delay90/1(d)
  Convert11/1 -> Delay100/1(d)
  Delay90/1(q) -> highmark2_23/1(out_high2)
  Delay100/1(q) -> highmark2_23/2(out_high3)
  delay22/1 -> highwater9/1(reset)
  delay71/1 -> highwater9/3(data)
  delay72/1 -> highwater9/2(valid)
  Constant15/1 -> Relational9/2
  Relational9/1 -> Logical25/2
  Logical25/1 -> delay60/1
  delay23/1 -> highwater8/1(reset)
  delay26/1 -> highwater8/3(data)
  delay60/1 -> highwater8/2(valid)
  highwater8/1(highmark) -> Convert15/1
  Constant17/1 -> Relational10/2
  Relational10/1 -> Logical26/2
  Logical26/1 -> delay69/1
  delay68/1 -> highwater11/3(data)
  delay69/1 -> highwater11/2(valid)
  Slice18/1 -> delay71/1, delay68/1, delay66/1, delay26/1
  Constant18/1 -> Relational11/2
  Relational11/1 -> Logical27/2
  Logical27/1 -> delay67/1
  [pre_valid_2] -> Logical23/1, Logical25/1, Logical27/1, Logical26/1
  delay64/1 -> highwater10/1(reset)
  delay66/1 -> highwater10/3(data)
  delay67/1 -> highwater10/2(valid)
  [cnt_rst] -> delay22/1, delay64/1, delay70/1, delay23/1
  Slice30/1 -> Relational8/1, Relational9/1, Relational11/1, Relational10/1
  [id0] -> highwater9/4(xid), highwater8/4(xid), highwater10/4(xid), highwater11/4(xid)
  delay70/1 -> highwater11/1(reset)
  highwater11/1(highmark) -> Convert10/1
  highwater10/1(highmark) -> Convert11/1
  [pre_freq_3] -> Slice25/1
  Constant19/1 -> Relational12/2
  [pre_feng_id_3] -> Slice28/1
  Relational12/1 -> Logical16/2
  Logical16/1 -> delay85/1
  Convert27/1 -> Delay101/1(d)
  highwater13/1(highmark) -> Convert27/1
  Delay101/1(q) -> highmark3_01/1(out_high0)
  Convert28/1 -> Delay103/1(d)
  Delay103/1(q) -> highmark3_01/2(out_high1)
  Convert25/1 -> Delay104/1(d)
  Convert26/1 -> Delay105/1(d)
  Delay104/1(q) -> highmark3_23/1(out_high2)
  Delay105/1(q) -> highmark3_23/2(out_high3)
  delay73/1 -> highwater13/1(reset)
  delay84/1 -> highwater13/3(data)
  delay85/1 -> highwater13/2(valid)
  Constant20/1 -> Relational13/2
  Relational13/1 -> Logical17/2
  Logical17/1 -> delay77/1
  delay74/1 -> highwater12/1(reset)
  delay76/1 -> highwater12/3(data)
  delay77/1 -> highwater12/2(valid)
  highwater12/1(highmark) -> Convert28/1
  Constant13/1 -> Relational14/2
  Relational14/1 -> Logical18/2
  Logical18/1 -> delay82/1
  delay81/1 -> highwater15/3(data)
  delay82/1 -> highwater15/2(valid)
  Slice25/1 -> delay76/1, delay79/1, delay81/1, delay84/1
  Constant14/1 -> Relational15/2
  Relational15/1 -> Logical19/2
  Logical19/1 -> delay80/1
  [pre_valid_3] -> Logical18/1, Logical19/1, Logical17/1, Logical16/1
  delay78/1 -> highwater14/1(reset)
  delay79/1 -> highwater14/3(data)
  delay80/1 -> highwater14/2(valid)
  [cnt_rst] -> delay83/1, delay78/1, delay74/1, delay73/1
  Slice28/1 -> Relational14/1, Relational15/1, Relational13/1, Relational12/1
  [id1] -> highwater15/4(xid), highwater14/4(xid), highwater12/4(xid), highwater13/4(xid)
  delay83/1 -> highwater15/1(reset)
  highwater15/1(highmark) -> Convert25/1
  highwater14/1(highmark) -> Convert26/1
  [vacc_txd3] -> Concat4/2
  [vacc_txd2] -> Concat4/1
  [vacc_txvld3] -> Concat5/2
  [vacc_txvld2] -> Concat5/1
  [vacc_txeof3] -> Concat6/2
